simulink library "xbsIndex_r3"  (Simulink 6.1)
(part 2 of 4)

      mask prompts: num_branches "Number of Branches"; branch_length "Lengths of Branches"; explicit_period "Use Explicit Sample Period"; period "Sample Period  (use -1 to inherit first known input period)"; rst "Provide Reset Port"; en "Provide Enable Port"; dbl_ovrd "Override with Doubles"; show_param "---------------------- Show Implementation Parameters -----------------------------------------------------------------------------------"; mem_type "Memory Type"; pipeline "Pipeline to Greatest Extent Possible"; use_rpm "Use Placement Information for Core"; gen_core "Generate Core"; xl_area "FPGA Area [Slices, FFs, BRAMs, LUTs, IOBs, Emb. Mults, TBUFs]"; xl_use_area "Use Area Above For Estimation"
      mask help:
      | BLOCK IS OUT OF DATE.
      |
      | This block is from an outdated copy of the Xilinx Blockset. Please run xlUpdateModel('<model-name>') to update to the latest version.
      mask init:
      | [enPortNum,enPortStr,rstPortNum,rstPortStr] = xlport_en_rst(en,rst,3);
      | [designRoot, family, part, speed, package, simulinkPeriod, sysclkPeriod, dbl_ovrd, trimVbit] = xlSysgenSettings(gcb,1,0);
      | trimVbit=1;
      | [bg,fg] = xlcmap_r3('PayCore',dbl_ovrd);
      | iPos = get_param(gcb,'Position');
      | iWidth=iPos(3)-iPos(1); iHeight=iPos(4)-iPos(2);
      | iCx=iWidth/2;
      | iCy=iHeight/2;
      | [logoX, logoY] = xlogo(iPos);
      | 
      | % one time added for param list
      | latency = 1;
      | dblOvrd = dbl_ovrd;
      | useCore = 1;
      | precision0 = 1;
      | precision1 = 1;
      | explicitClk = explicit_period;
      | gen_core = 1;
      | rpm = use_rpm;
      | hasEN = en;
      | hasRST = rst;
      | % just pass everything to s-function
      | sfcn_mwsv__ = get_param(gcb, 'MaskWSVariables');
      | 
      | nport = get_param(gcbh, 'ports');
      | nin = nport(1);
      | nout = nport(2);
      mask Help: eval('xlWeb(xlhtmldoclink(''Interleaver Deinterleaver''))');
      mask StyleString: popup(Interleaver|Deinterleaver),edit,edit,checkbox,edit,checkbox,checkbox,checkbox,checkbox,popup(Automatically Chosen|Block RAM|Distributed RAM),checkbox,checkbox,checkbox,edit,checkbox
      mask Display:
      | patch([0 iWidth iWidth 0],[0 0 iHeight iHeight] , bg);
      | patch(logoX,logoY , fg);
      | port_label('input',1,'din');
      | port_label('output',1,'dout' );
      | port_label('output',2,'vout');
      | port_label('input',2,'vin');
      | port_label('input',enPortNum,enPortStr);
      | port_label('input',rstPortNum,rstPortStr);
      | plot([0 0 iWidth iWidth 0], [0 iHeight iHeight 0 0]);
  Inverter : S-Function  FunctionName=xldeprecated  Parameters=nin,nout  mask(Xilinx Inverter){latency=0, explicit_period=off, period=1, en=off, dbl_ovrd=off, show_param=off, xl_area=[0, 0, 0, 0, 0, 0, 0], xl_use_area=off}
      mask prompts: explicit_period "Use Explicit Sample Period"; period "Sample Period  (use -1 to inherit first known input period)"; en "Provide Enable Port"; dbl_ovrd "Override with Doubles"; show_param "---------------------- Show Implementation Parameters -----------------------------------------------------------------------------------"; xl_area "FPGA Area [Slices, FFs, BRAMs, LUTs, IOBs, Emb. Mults, TBUFs]"; xl_use_area "Use Area Above For Estimation"
      mask help:
      | BLOCK IS OUT OF DATE.
      |
      | This block is from an outdated copy of the Xilinx Blockset. Please run xlUpdateModel('<model-name>') to update to the latest version.
      mask init:
      | [enPortNum,enPortStr] = xlport_en_rst(en,0,2);
      | 
      | [designRoot, family, part, speed, package, simulinkPeriod, sysclkPeriod, dbl_ovrd, trimVbit] = xlSysgenSettings(gcb,1,1);
      | zstr=''; zpstr='';
      | if latency > 0
      |   zstr = 'z';
      |   zpstr = sprintf('-%d', latency);
      | end
      | [bg,fg] = xlcmap_r3('XBlock',dbl_ovrd);
      | iPos = get_param(gcb,'Position');
      | iWidth=iPos(3)-iPos(1); iHeight=iPos(4)-iPos(2);
      | iCx=iWidth/2;
      | iCy=iHeight/2;
      | [logoX, logoY] = xlogo(iPos);
      | zstrx = 0.45*iWidth-3; if (zstrx<3) zstrx=3; end
      | zstry = 0.36*iHeight-7; if (zstry<3) zstry=3; end
      | 
      | 
      | 
      | % one time added for param list
      | dblOvrd = dbl_ovrd;
      | precision0 = 1;
      | explicitClk = explicit_period;
      | 
      | hasEN = en;
      | 
      | % just pass everything to s-function
      | sfcn_mwsv__ = get_param(gcb, 'MaskWSVariables');
      | 
      | nport = get_param(gcbh, 'ports');
      | nin = nport(1);
      | nout = nport(2);
      mask Help: eval('xlWeb(xlhtmldoclink(''Inverter''))');
      mask Display:
      | patch([0 iWidth iWidth 0],[0 0 iHeight iHeight] , bg);
      | patch(logoX,logoY, fg);
      | text(zstrx,zstry,zstr);
      | text(zstrx+5,zstry+5,zpstr);
      | disp(' not');
      | port_label('input',enPortNum,enPortStr);
      | ;plot([0 0 iWidth iWidth 0], [0 iHeight iHeight 0 0]);
  J.83 Modulator : S-Function  FunctionName=xldeprecated  Parameters=nin,nout  mask(J.83 Modulator){}
      mask help:
      | BLOCK IS OUT OF DATE.
      |
      | This block is from an outdated copy of the Xilinx Blockset. Please run xlUpdateModel('<model-name>') to update to the latest version.
      mask init:
      | % Set Block Logo
      | [bg,fg] = xlcmap_r3('PayCore',0);
      | iPos = get_param(gcb,'Position');
      | iWidth=iPos(3)-iPos(1); iHeight=iPos(4)-iPos(2);
      | iCx=iWidth/2;
      | iCy=iHeight/2;
      | [logoX, logoY] = xlogo(iPos);
      | 
      | errormsg = ['This block has not yet been installed.  You may download this and other blocks from the Xilinx web site by clicking on the block help button.'];
      | num_inports = 0;
      | num_outports = 0;
      | nport = get_param(gcbh, 'ports');
      | nin = nport(1);
      | nout = nport(2);
      mask Help: eval('xlWeb(xlhtmldoclink(''J.83 Modulator''))');
      mask Display:
      | patch([0 iWidth iWidth 0],[0 0 iHeight iHeight] , bg);
      | patch(logoX,logoY, fg);
      | text(iCx-29,iCy,'Not Installed');
      | plot([0 0 iWidth iWidth 0], [0 iHeight iHeight 0 0]);
  LFSR : S-Function  FunctionName=xldeprecated  Parameters=nin,nout  mask(Xilinx Linear Feedback Shift Register){lfsr_type=Fibonacci, gate_type=XOR, output_type=off, n_bits=6, bin_pt=4, arith_type=Unsigned, polynomial='11', rst_value='3F', reloadable_seed=off, input_type=off, explicit_period=on, period=1, rst=off, en=off, dbl_ovrd=off, show_param=off, useSRL16s=off, use_rpm=off, gen_core=off, xl_area=[0, 0, 0, 0, 0, 0, 0], xl_use_area=off}
      mask prompts: lfsr_type "Type"; gate_type "Gate Type"; output_type "Parallel Output"; n_bits "Number of Bits in LFSR"; bin_pt "Binary Point Position"; arith_type "Arithmetic Type"; polynomial "Feedback Polynomial (Enter hex value enclosed with ticks)"; rst_value "Initial Value (Enter hex value enclosed with ticks)"; reloadable_seed "Use Reloadable Seed Values"; input_type "Parallel Input"; explicit_period "Use Explicit Sample Period"; period "Sample Period"; rst "Provide Reset Port"; en "Provide Enable Port"; dbl_ovrd "Override with Doubles"; show_param "---------------------- Show Implementation Parameters -----------------------------------------------------------------------------------"; useSRL16s "Implement with SRL16s"; use_rpm "Use Placement Information for Core"; gen_core "Generate Core"; xl_area "FPGA Area [Slices, FFs, BRAMs, LUTs, IOBs, Emb. Mults, TBUFs]"; xl_use_area "Use Area Above For Estimation"
      mask help:
      | BLOCK IS OUT OF DATE.
      |
      | This block is from an outdated copy of the Xilinx Blockset. Please run xlUpdateModel('<model-name>') to update to the latest version.
      mask init:
      | numinputs = 1;
      | dinDir = 'output';
      | dinPNum = 1;
      | dinStr = '';
      | loadDir = 'output';
      | loadPNum = 1;
      | loadStr = '';
      | 
      | if (reloadable_seed)
      |    dinStr = 'din';
      |    dinDir = 'input';
      |    dinPNum = 1;
      |    loadStr = 'load';
      |    loadDir = 'input';
      |    loadPNum = 2;
      |    numinputs = numinputs + 2;
      | end
      | 
      | [enPortNum, enPortStr, rstPortNum, rstPortStr, portDir] = xlport_en_rst(en, rst, numinputs);
      | 
      | [designRoot, family, part, speed, package, simulinkPeriod, sysclkPeriod, dbl_ovrd, trimVbit] = xlSysgenSettings(gcb,1,1);
      | [bg,fg]=xlcmap_r3('XBlock',dbl_ovrd);
      | iPos = get_param(gcb,'Position');
      | iWidth=iPos(3)-iPos(1); iHeight=iPos(4)-iPos(2);
      | iCx=iWidth/2;
      | iCy=iHeight/2;
      | [logoX, logoY] = xlogo(iPos);
      | 
      | 
      | % one time added for param list
      | dblOvrd = dbl_ovrd;
      | precision0 = 2;
      | z0 = [n_bits bin_pt arith_type  1 1];
      | hasEN = en;
      | hasRST = rst;
      | latency = 1;
      | useCore = 1;
      | explicitClk = explicit_period;
      | gen_core = 1;
      | % just pass everything to s-function
      | sfcn_mwsv__ = get_param(gcb, 'MaskWSVariables');
      | 
      | nport = get_param(gcbh, 'ports');
      | nin = nport(1);
      | nout = nport(2);
      mask Help: eval('xlWeb(xlhtmldoclink(''LFSR''))');
      mask StyleString: popup(Fibonacci|Galois),popup(XOR|XNOR),checkbox,edit,edit,popup(Unsigned|Signed  (2's comp)),edit,edit,checkbox,checkbox,checkbox,edit,checkbox,checkbox,checkbox,checkbox,checkbox,checkbox,checkbox,edit,checkbox
      mask Display:
      | patch([0 iWidth iWidth 0],[0 0 iHeight iHeight] , bg);
      | patch(logoX,logoY , fg);
      | port_label('output',1,'dout');
      | port_label(dinDir,dinPNum,dinStr);
      | port_label(loadDir,loadPNum,loadStr);
      | port_label(portDir,rstPortNum,rstPortStr);
      | port_label(portDir,enPortNum,enPortStr);
      | plot([0 0 iWidth iWidth 0], [0 iHeight iHeight 0 0]);
  Logical : S-Function  FunctionName=xldeprecated  Parameters=nin,nout  mask(Xilinx Logical Block){logical_function=AND, inputs=2, precision=Full, arith_type=Unsigned, n_bits=8, bin_pt=2, align_bp=on, latency=0, explicit_period=off, period=1, en=off, dbl_ovrd=off, show_param=off, xl_area=[0, 0, 0, 0, 0, 0, 0], xl_use_area=off}
      mask prompts: logical_function "Logical Function"; inputs "Number of Inputs"; arith_type "Output Type"; n_bits "Number of Bits"; bin_pt "Binary Point"; align_bp "Align Binary Point"; explicit_period "Use Explicit Sample Period"; period "Sample Period  (use -1 to inherit first known input period)"; en "Provide Enable Port"; dbl_ovrd "Override with Doubles"; show_param "---------------------- Show Implementation Parameters -----------------------------------------------------------------------------------"; xl_area "FPGA Area [Slices, FFs, BRAMs, LUTs, IOBs, Emb. Mults, TBUFs]"; xl_use_area "Use Area Above For Estimation"
      mask help:
      | BLOCK IS OUT OF DATE.
      |
      | This block is from an outdated copy of the Xilinx Blockset. Please run xlUpdateModel('<model-name>') to update to the latest version.
      mask init:
      | [enPortNum,enPortStr] = xlport_en_rst(en,0,inputs+2);
      | 
      | num_inputs = inputs+1;
      | [designRoot, family, part, speed, package, simulinkPeriod, sysclkPeriod, dbl_ovrd, trimVbit] = xlSysgenSettings(gcb,1,1);
      | operators = [' and'; 'nand'; '  or'; ' nor'; ' xor'; 'xnor'];
      | ostr = operators(logical_function,1:4);
      | [bg,fg] = xlcmap_r3('XBlock',dbl_ovrd);
      | iPos = get_param(gcb,'Position');
      | iWidth=iPos(3)-iPos(1); iHeight=iPos(4)-iPos(2);
      | iCx=iWidth/2;
      | iCy=iHeight/2;
      | [logoX, logoY] = xlogo(iPos);
      | zstr=''; zpstr='';
      | if latency > 0
      |   zstr = 'z';
      |   zpstr = sprintf('-%d', latency);
      | end
      | zstrx = 0.45*iWidth-3; if (zstrx<3) zstrx=3; end
      | zstry = 0.36*iHeight-7; if (zstry<3) zstry=3; end
      | 
      | % one time added for param list
      | dblOvrd = dbl_ovrd;
      | numInputs = num_inputs;
      | precision0 = precision;
      | z0 = [n_bits bin_pt arith_type 1 1 ];
      | explicitClk = explicit_period;
      | hasEN = en;
      | 
      | % just pass everything to s-function
      | sfcn_mwsv__ = get_param(gcb, 'MaskWSVariables');
      | 
      | nport = get_param(gcbh, 'ports');
      | nin = nport(1);
      | nout = nport(2);
      mask Help: eval('xlWeb(xlhtmldoclink(''Logical''))');
      mask StyleString: popup(AND|NAND|OR|NOR|XOR|XNOR),popup(2|3|4),popup(Full|User Defined),popup(Unsigned|Signed  (2's comp)),edit,edit,checkbox,edit,checkbox,edit,checkbox,checkbox,checkbox,edit,checkbox
      mask Display:
      | patch([0 iWidth iWidth 0],[0 0 iHeight iHeight] ,bg);
      | patch(logoX,logoY,  fg);
      | text(zstrx,zstry,zstr);
      | text(zstrx+5,zstry+5,zpstr);
      | disp(ostr);
      | ;plot([0 0 iWidth iWidth 0], [0 iHeight iHeight 0 0]);
      | port_label('input',enPortNum,enPortStr);
  MCode : S-Function  FunctionName=xldeprecated  Parameters=nin,nout  mask(Xilinx MCode Block){mfname=xlmax, defparams={}, suppress_output=off, hide_port_list={}, explicit_period=off, period=1, dbl_ovrd=off, show_param=off, xl_area=[0, 0, 0, 0, 0, 0, 0], xl_use_area=off}
      mask prompts: mfname "MATLAB Function"; defparams "Function Parameter Bindings (cell array, e.g., {'name', value, ...})"; suppress_output "Suppress Selected Output Ports"; hide_port_list "Output Ports to Suppress (cell array, e.g., {'name1', 'name2', ...})"; explicit_period "Use Explicit Sample Period"; period "Sample Period  (use -1 to inherit first known input period)"; dbl_ovrd "Override with Doubles"; show_param "---------------------- Show Implementation Parameters -----------------------------------------------------------------------------------"; xl_area "FPGA Area (slice, FF, BRAM, LUT, IOB, Hard Mults, TBUF)"; xl_use_area "Use Area Above For Estimation"
      mask help:
      | BLOCK IS OUT OF DATE.
      |
      | This block is from an outdated copy of the Xilinx Blockset. Please run xlUpdateModel('<model-name>') to update to the latest version.
      mask init:
      | %remove these!
      | use_rpm = 0;
      | use_core = 0;
      | clear xlmcode_maskinit;
      | if ~suppress_output
      | 	hide_port_list = {};
      | end
      | mfilename = xlFindMFile(mfname);
      | [param_names_double, param_values_double, param_names_bool, param_values_bool, error_msgs] = xlmcode_parsedefparam(defparams);
      | [numin, innums, inports, numout, outnums, outports, inname, outname] = xlmcode_maskinit(mfilename, 128, param_names_double, param_values_double, param_names_bool, param_values_bool, hide_port_list);
      | 
      | if numin==0
      |   explicitClk = 1;
      | else
      |   explicitClk = explicit_period;
      | end
      | 
      | blk = gcb;
      | visstr = get_param(blk,'MaskVisibilities');
      | var = get_param(blk,'MaskNames');
      | 
      | explicit_period_pos = find(strcmp(var,'explicit_period'));
      | period_pos = find(strcmp(var,'period'));
      | if numin==0
      |   % we need to hide the explicit_period parameter and show period
      |   visstr(explicit_period_pos) = {'off'};
      |   visstr(period_pos) = {'on'};
      | else
      |   visstr(explicit_period_pos) = {'on'};
      |   if explicit_period
      |     visstr(period_pos) = {'on'};
      |   else
      |     visstr(period_pos) = {'off'};
      |   end
      | end
      | 
      | set_param(blk, 'MaskVisibilities', visstr);
      | 
      | [designRoot, family, part, speed, package, simulinkPeriod, sysclkPeriod, dbl_ovrd, trimVbit] = xlSysgenSettings(gcb,1,1);
      | [bg,fg] = xlcmap_r3('XBlock',dbl_ovrd);
      | iPos = get_param(gcb,'Position');
      | iWidth=iPos(3)-iPos(1); iHeight=iPos(4)-iPos(2);
      | iCx=iWidth/2;
      | iCy=iHeight/2;
      | [logoX, logoY] = xlogo(iPos);
      | zstr=''; zpstr='';
      | zstr = mfname;
      | zstrx = 0.50*iWidth-3-length(mfname); if (zstrx<3) zstrx=3; end
      | zstry = 0.40*iHeight+6; if (zstry<3) zstry=3; end
      | 
      | % one time added for param list
      | latency = 0;
      | dblOvrd = dbl_ovrd;
      | numInputs = numin;
      | useCore = use_core;
      | precision0 = 1;
      | z0 = [1 0 1 1 1 ];
      | precision1 = 1;
      | precision2 = 1;
      | precision3 = 1;
      | precision4 = 1;
      | precision5 = 1;
      | precision6 = 1;
      | precision7 = 1;
      | precision8 = 1;
      | precision9 = 1;
      | precision10 = 1;
      | precision11 = 1;
      | precision12 = 1;
      | precision13 = 1;
      | precision14 = 1;
      | precision15 = 1;
      | 
      | rpm = use_rpm;
      | 
      | % mwsv_list = {'mfilename', 'designRoot', 'family', 'part', 'speed', 'package', 'simulinkPeriod', 'sysclkPeriod', 'latency', 'dblOvrd', 'trimVbit', 'numInputs', 'numout', 'useCore', 'precision0', 'z0', 'explicitClk', 'param_names_double', 'param_values_double', 'param_names_bool', 'param_values_bool', 'hide_port_list', 'period'};
      | % just pass everything to s-function
      | sfcn_mwsv__ = xlfiltermwsv(get_param(gcb, 'MaskWSVariables'), {'defparams'});
      | 
      | nport = get_param(gcbh, 'ports');
      | nin = nport(1);
      | nout = nport(2);
      mask Help: eval('xlWeb(xlhtmldoclink(''MCode''))');
      mask Display:
      | patch([0 iWidth iWidth 0],[0 0 iHeight iHeight] ,bg);
      | patch(logoX,logoY,  fg);
      | disp(mfname);
      | 
      | ;plot([0 0 iWidth iWidth 0], [0 iHeight iHeight 0 0]);
      | 
      | port_label(inname, innums(1), inports{1});
      | port_label(inname, innums(2), inports{2});
      | port_label(inname, innums(3), inports{3});
      | port_label(inname, innums(4), inports{4});
      | port_label(inname, innums(5), inports{5});
      | port_label(inname, innums(6), inports{6});
      | port_label(inname, innums(7), inports{7});
      | port_label(inname, innums(8), inports{8});
      | port_label(inname, innums(9), inports{9});
      | port_label(inname, innums(10), inports{10});
      | port_label(inname, innums(11), inports{11});
      | port_label(inname, innums(12), inports{12});
      | port_label(inname, innums(13), inports{13});
      | port_label(inname, innums(14), inports{14});
      | port_label(inname, innums(15), inports{15});
      | port_label(inname, innums(16), inports{16});
      | port_label(inname, innums(17), inports{17});
      | port_label(inname, innums(18), inports{18});
      | port_label(inname, innums(19), inports{19});
      | port_label(inname, innums(20), inports{20});
      | port_label(inname, innums(21), inports{21});
      | port_label(inname, innums(22), inports{22});
      | port_label(inname, innums(23), inports{23});
      | port_label(inname, innums(24), inports{24});
      | port_label(inname, innums(25), inports{25});
      | port_label(inname, innums(26), inports{26});
      | port_label(inname, innums(27), inports{27});
      | port_label(inname, innums(28), inports{28});
      | port_label(inname, innums(29), inports{29});
      | port_label(inname, innums(30), inports{30});
      | port_label(inname, innums(31), inports{31});
      | port_label(inname, innums(32), inports{32});
      | port_label(inname, innums(33), inports{33});
      | port_label(inname, innums(34), inports{34});
      | port_label(inname, innums(35), inports{35});
      | port_label(inname, innums(36), inports{36});
      | port_label(inname, innums(37), inports{37});
      | port_label(inname, innums(38), inports{38});
      | port_label(inname, innums(39), inports{39});
      | port_label(inname, innums(40), inports{40});
      | port_label(inname, innums(41), inports{41});
      | port_label(inname, innums(42), inports{42});
      | port_label(inname, innums(43), inports{43});
      | port_label(inname, innums(44), inports{44});
      | port_label(inname, innums(45), inports{45});
      | port_label(inname, innums(46), inports{46});
      | port_label(inname, innums(47), inports{47});
      | port_label(inname, innums(48), inports{48});
      | port_label(inname, innums(49), inports{49});
      | port_label(inname, innums(50), inports{50});
      | port_label(inname, innums(51), inports{51});
      | port_label(inname, innums(52), inports{52});
      | port_label(inname, innums(53), inports{53});
      | port_label(inname, innums(54), inports{54});
      | port_label(inname, innums(55), inports{55});
      | port_label(inname, innums(56), inports{56});
      | port_label(inname, innums(57), inports{57});
      | port_label(inname, innums(58), inports{58});
      | port_label(inname, innums(59), inports{59});
      | port_label(inname, innums(60), inports{60});
      | port_label(inname, innums(61), inports{61});
      | port_label(inname, innums(62), inports{62});
      | port_label(inname, innums(63), inports{63});
      | port_label(inname, innums(64), inports{64});
      | port_label(inname, innums(65), inports{65});
      | port_label(inname, innums(66), inports{66});
      | port_label(inname, innums(67), inports{67});
      | port_label(inname, innums(68), inports{68});
      | port_label(inname, innums(69), inports{69});
      | port_label(inname, innums(70), inports{70});
      | port_label(inname, innums(71), inports{71});
      | port_label(inname, innums(72), inports{72});
      | port_label(inname, innums(73), inports{73});
      | port_label(inname, innums(74), inports{74});
      | port_label(inname, innums(75), inports{75});
      | port_label(inname, innums(76), inports{76});
      | port_label(inname, innums(77), inports{77});
      | port_label(inname, innums(78), inports{78});
      | port_label(inname, innums(79), inports{79});
      | port_label(inname, innums(80), inports{80});
      | port_label(inname, innums(81), inports{81});
      | port_label(inname, innums(82), inports{82});
      | port_label(inname, innums(83), inports{83});
      | port_label(inname, innums(84), inports{84});
      | port_label(inname, innums(85), inports{85});
      | port_label(inname, innums(86), inports{86});
      | port_label(inname, innums(87), inports{87});
      | port_label(inname, innums(88), inports{88});
      | port_label(inname, innums(89), inports{89});
      | port_label(inname, innums(90), inports{90});
      | port_label(inname, innums(91), inports{91});
      | port_label(inname, innums(92), inports{92});
      | port_label(inname, innums(93), inports{93});
      | port_label(inname, innums(94), inports{94});
      | port_label(inname, innums(95), inports{95});
      | port_label(inname, innums(96), inports{96});
      | port_label(inname, innums(97), inports{97});
      | port_label(inname, innums(98), inports{98});
      | port_label(inname, innums(99), inports{99});
      | port_label(inname, innums(100), inports{100});
      | port_label(inname, innums(101), inports{101});
      | port_label(inname, innums(102), inports{102});
      | port_label(inname, innums(103), inports{103});
      | port_label(inname, innums(104), inports{104});
      | port_label(inname, innums(105), inports{105});
      | port_label(inname, innums(106), inports{106});
      | port_label(inname, innums(107), inports{107});
      | port_label(inname, innums(108), inports{108});
      | port_label(inname, innums(109), inports{109});
      | port_label(inname, innums(110), inports{110});
      | port_label(inname, innums(111), inports{111});
      | port_label(inname, innums(112), inports{112});
      | port_label(inname, innums(113), inports{113});
      | port_label(inname, innums(114), inports{114});
      | port_label(inname, innums(115), inports{115});
      | port_label(inname, innums(116), inports{116});
      | port_label(inname, innums(117), inports{117});
      | port_label(inname, innums(118), inports{118});
      | port_label(inname, innums(119), inports{119});
      | port_label(inname, innums(120), inports{120});
      | port_label(inname, innums(121), inports{121});
      | port_label(inname, innums(122), inports{122});
      | port_label(inname, innums(123), inports{123});
      | port_label(inname, innums(124), inports{124});
      | port_label(inname, innums(125), inports{125});
      | port_label(inname, innums(126), inports{126});
      | port_label(inname, innums(127), inports{127});
      | port_label(inname, innums(128), inports{128});
      | 
      | port_label(outname, outnums(1), outports{1});
      | port_label(outname, outnums(2), outports{2});
      | port_label(outname, outnums(3), outports{3});
      | port_label(outname, outnums(4), outports{4});
      | port_label(outname, outnums(5), outports{5});
      | port_label(outname, outnums(6), outports{6});
      | port_label(outname, outnums(7), outports{7});
      | port_label(outname, outnums(8), outports{8});
      | port_label(outname, outnums(9), outports{9});
      | port_label(outname, outnums(10), outports{10});
      | port_label(outname, outnums(11), outports{11});
      | port_label(outname, outnums(12), outports{12});
      | port_label(outname, outnums(13), outports{13});
      | port_label(outname, outnums(14), outports{14});
      | port_label(outname, outnums(15), outports{15});
      | port_label(outname, outnums(16), outports{16});
      | port_label(outname, outnums(17), outports{17});
      | port_label(outname, outnums(18), outports{18});
      | port_label(outname, outnums(19), outports{19});
      | port_label(outname, outnums(20), outports{20});
      | port_label(outname, outnums(21), outports{21});
      | port_label(outname, outnums(22), outports{22});
      | port_label(outname, outnums(23), outports{23});
      | port_label(outname, outnums(24), outports{24});
      | port_label(outname, outnums(25), outports{25});
      | port_label(outname, outnums(26), outports{26});
      | port_label(outname, outnums(27), outports{27});
      | port_label(outname, outnums(28), outports{28});
      | port_label(outname, outnums(29), outports{29});
      | port_label(outname, outnums(30), outports{30});
      | port_label(outname, outnums(31), outports{31});
      | port_label(outname, outnums(32), outports{32});
      | port_label(outname, outnums(33), outports{33});
      | port_label(outname, outnums(34), outports{34});
      | port_label(outname, outnums(35), outports{35});
      | port_label(outname, outnums(36), outports{36});
      | port_label(outname, outnums(37), outports{37});
      | port_label(outname, outnums(38), outports{38});
      | port_label(outname, outnums(39), outports{39});
      | port_label(outname, outnums(40), outports{40});
      | port_label(outname, outnums(41), outports{41});
      | port_label(outname, outnums(42), outports{42});
      | port_label(outname, outnums(43), outports{43});
      | port_label(outname, outnums(44), outports{44});
      | port_label(outname, outnums(45), outports{45});
      | port_label(outname, outnums(46), outports{46});
      | port_label(outname, outnums(47), outports{47});
      | port_label(outname, outnums(48), outports{48});
      | port_label(outname, outnums(49), outports{49});
      | port_label(outname, outnums(50), outports{50});
      | port_label(outname, outnums(51), outports{51});
      | port_label(outname, outnums(52), outports{52});
      | port_label(outname, outnums(53), outports{53});
      | port_label(outname, outnums(54), outports{54});
      | port_label(outname, outnums(55), outports{55});
      | port_label(outname, outnums(56), outports{56});
      | port_label(outname, outnums(57), outports{57});
      | port_label(outname, outnums(58), outports{58});
      | port_label(outname, outnums(59), outports{59});
      | port_label(outname, outnums(60), outports{60});
      | port_label(outname, outnums(61), outports{61});
      | port_label(outname, outnums(62), outports{62});
      | port_label(outname, outnums(63), outports{63});
      | port_label(outname, outnums(64), outports{64});
      | port_label(outname, outnums(65), outports{65});
      | port_label(outname, outnums(66), outports{66});
      | port_label(outname, outnums(67), outports{67});
      | port_label(outname, outnums(68), outports{68});
      | port_label(outname, outnums(69), outports{69});
      | port_label(outname, outnums(70), outports{70});
      | port_label(outname, outnums(71), outports{71});
      | port_label(outname, outnums(72), outports{72});
      | port_label(outname, outnums(73), outports{73});
      | port_label(outname, outnums(74), outports{74});
      | port_label(outname, outnums(75), outports{75});
      | port_label(outname, outnums(76), outports{76});
      | port_label(outname, outnums(77), outports{77});
      | port_label(outname, outnums(78), outports{78});
      | port_label(outname, outnums(79), outports{79});
      | port_label(outname, outnums(80), outports{80});
      | port_label(outname, outnums(81), outports{81});
      | port_label(outname, outnums(82), outports{82});
      | port_label(outname, outnums(83), outports{83});
      | port_label(outname, outnums(84), outports{84});
      | port_label(outname, outnums(85), outports{85});
      | port_label(outname, outnums(86), outports{86});
      | port_label(outname, outnums(87), outports{87});
      | port_label(outname, outnums(88), outports{88});
      | port_label(outname, outnums(89), outports{89});
      | port_label(outname, outnums(90), outports{90});
      | port_label(outname, outnums(91), outports{91});
      | port_label(outname, outnums(92), outports{92});
      | port_label(outname, outnums(93), outports{93});
      | port_label(outname, outnums(94), outports{94});
      | port_label(outname, outnums(95), outports{95});
      | port_label(outname, outnums(96), outports{96});
      | port_label(outname, outnums(97), outports{97});
      | port_label(outname, outnums(98), outports{98});
      | port_label(outname, outnums(99), outports{99});
      | port_label(outname, outnums(100), outports{100});
      | port_label(outname, outnums(101), outports{101});
      | port_label(outname, outnums(102), outports{102});
      | port_label(outname, outnums(103), outports{103});
      | port_label(outname, outnums(104), outports{104});
      | port_label(outname, outnums(105), outports{105});
      | port_label(outname, outnums(106), outports{106});
      | port_label(outname, outnums(107), outports{107});
      | port_label(outname, outnums(108), outports{108});
      | port_label(outname, outnums(109), outports{109});
      | port_label(outname, outnums(110), outports{110});
      | port_label(outname, outnums(111), outports{111});
      | port_label(outname, outnums(112), outports{112});
      | port_label(outname, outnums(113), outports{113});
      | port_label(outname, outnums(114), outports{114});
      | port_label(outname, outnums(115), outports{115});
      | port_label(outname, outnums(116), outports{116});
      | port_label(outname, outnums(117), outports{117});
      | port_label(outname, outnums(118), outports{118});
      | port_label(outname, outnums(119), outports{119});
      | port_label(outname, outnums(120), outports{120});
      | port_label(outname, outnums(121), outports{121});
      | port_label(outname, outnums(122), outports{122});
      | port_label(outname, outnums(123), outports{123});
      | port_label(outname, outnums(124), outports{124});
      | port_label(outname, outnums(125), outports{125});
      | port_label(outname, outnums(126), outports{126});
      | port_label(outname, outnums(127), outports{127});
      | port_label(outname, outnums(128), outports{128});
  MicroBlaze Processor : Subsystem  mask(MicroBlaze Processor){t__general=0, in_if=1, in_depths=32, out_if=1, out_depths=32, async=on, rstport=off, paramchksum=1:1:32:32:on:off:off:<empty>, procmodel=off, t__hardware=0, hw_hwcosimmodel=<empty>, hw_addsimmodel=0, t__software=0, sw_editsrccode=0ffgd, sw_compsrccode=0, xlBlockVersion=6.3}
      mask prompts: t__general "::General"; in_if "Number of Input Interfaces"; in_depths "Input FIFO Depths"; out_if "Number of Output Interfaces"; out_depths "Output FIFO Depths"; async "Use Asynchronous FIFOs"; rstport "Provide Reset Port"; paramchksum "paramchecksum"; procmodel "Provide Processor Model"; t__hardware "::Hardware"; hw_hwcosimmodel "Simulation Model"; hw_addsimmodel ":button:Add Simulation Model"; t__software "::Software"; sw_editsrccode ":button:Edit Source Code"; sw_compsrccode ":button:Compile Source Code"
      mask help:
      | Provides a MicroBlaze stub for designing peripherals that communicate with the processor using Fast Simplex Links (FSL). Current MicroBlaze implementation allows a maximum of  8 input and 8 output ports.
      |
      | Select 'Provide Processor Model' to enable use of hardware co-simulation models.
      mask init:
      | [bg,fg] = xlcmap_r3('XBlock',0);
      | iPos = get_param(gcb,'Position');
      | iWidth=iPos(3)-iPos(1); iHeight=iPos(4)-iPos(2);
      | iCx=iWidth/2;
      | iCy=iHeight/2;
      | [logoX, logoY] = xlogo(iPos);
      | [xldirectory, xlSynthTool] = xlFindTargetDir(gcb);
      | 
      | if (~strcmp(bdroot(gcs),'xbsControl_r3'))
      | 	set_param(gcb, 'LinkStatus', 'none');
      | 	xlMBCallbacks('initSubsystem');
      | end;
      settings: OpenFcn=modelName = get_param(bdroot, 'name');h = errordlg(sprintf(['This block is from an outdated copy of the Xilinx Blockset.\nPlease run xlUpdateModel(''' modelName ''') to update this design.']), 'Update Required');
      mask Help: eval('xlWeb(xlhtmldoclink(''MicroBlaze Processor''))');
      mask StyleString: edit,edit,edit,edit,edit,checkbox,checkbox,edit,checkbox,edit,popup(<empty>),edit,edit,edit,edit,edit
      mask Display:
      | patch([0 iWidth iWidth 0],[0 0 iHeight iHeight] , bg);patch(logoX,logoY , fg);plot([0 0 iWidth iWidth 0], [0 iHeight iHeight 0 0]);disp('Stub');
      | port_label('input',1,'In0_data');
      | port_label('input',2,'In0_control');
      | port_label('input',3,'In0_write');
      | port_label('input',4,'Out0_read');
      | port_label('output',1,'In0_full');
      | port_label('output',2,'Out0_data');
      | port_label('output',3,'Out0_control');
      | port_label('output',4,'Out0_exists');
  ModelSim : S-Function  FunctionName=xldeprecated  Parameters=nin,nout  mask(ModelSim HDL Co-Simulation Interface){dir=./modelsim, waveform=on, leave_open=on, skip_compile=off, custom_scripts=off, pre_comp_script=, vsim_script=, post_vsim_script=, startup_timeout=40}
      mask prompts: dir "Run Co-Simulation in Directory:"; waveform "Open Waveform Viewer"; leave_open "Leave ModelSim Open at End of Simulation"; skip_compile "Skip Compilation  (use previous results )"; custom_scripts "Add Custom Scripts"; pre_comp_script "Script to Run Before Starting Compilation:"; vsim_script "Script to Run in Place of  "vsim":"; post_vsim_script "Script to Run After "vsim":"
      mask help:
      | BLOCK IS OUT OF DATE.
      |
      | This block is from an outdated copy of the Xilinx Blockset. Please run xlUpdateModel('<model-name>') to update to the latest version.
      mask init:
      | engineDLL = 'MTICosimEng.dll';
      | binDir = xlPathToReference;
      | 
      | sim_status = get_param(bdroot,'SimulationStatus');
      | 
      | [bg,fg] = xlcmap_r3('XTool');
      | 
      | iPos = get_param(gcb,'Position');
      | iWidth=iPos(3)-iPos(1); iHeight=iPos(4)-iPos(2);
      | iCx=iWidth/2;
      | iCy=iHeight/2;
      | [logoX, logoY] = xlogo(iPos);
      | 
      | [mdlPath mdlFile mdlExt] = fileparts(get_param(bdroot,'filename'));
      | 
      | screenSize = get(0,'screensize');
      | screenSize = screenSize([3 4]);
      | 
      | % just pass everything to s-function
      | sfcn_mwsv__ = get_param(gcb, 'MaskWSVariables');
      | 
      | nport = get_param(gcbh, 'ports');
      | nin = nport(1);
      | nout = nport(2);
      mask Help: eval('xlWeb(xlhtmldoclink(''ModelSim''))');
      mask Display:
      | patch([0 iWidth iWidth 0],[0 0 iHeight iHeight] , bg);
      | patch(logoX,logoY, fg);
      | plot([0 0 iWidth iWidth 0], [0 iHeight iHeight 0 0]);
      | text(6,iHeight-11,'ModelSim');
  Mult : S-Function  FunctionName=xldeprecated  Parameters=nin,nout  mask(Xilinx Multiplier){precision=Full, arith_type=Signed  (2's comp), n_bits=8, bin_pt=2, quantization=Truncate, overflow=Wrap, latency=3, explicit_period=off, period=1, en=off, dbl_ovrd=off, show_param=off, mult_type=Parallel, oversample=2, use_embedded=off, pipeline=on, use_rpm=on, placement_style=Rectangular Shape, gen_core=off, xl_area=[0, 0, 0, 0, 0, 0, 0], xl_use_area=off}
      mask prompts: arith_type "Output Type"; n_bits "Number of Bits"; bin_pt "Binary Point"; explicit_period "Use Explicit Sample Period"; period "Sample Period  (use -1 to inherit first known input period)"; en "Provide Enable Port"; dbl_ovrd "Override with Doubles"; show_param "---------------------- Show Implementation Parameters -----------------------------------------------------------------------------------"; mult_type "Multiplier Type"; oversample "Hardware Over-Sampling Rate"; use_embedded "Use Embedded Multipliers"; pipeline "Pipeline to Greatest Extent Possible"; use_rpm "Use Placement Information for Core"; placement_style "Placement Style"; gen_core "Generate Core"; xl_area "FPGA Area [Slices, FFs, BRAMs, LUTs, IOBs, Emb. Mults, TBUFs]"; xl_use_area "Use Area Above For Estimation"
      mask help:
      | BLOCK IS OUT OF DATE.
      |
      | This block is from an outdated copy of the Xilinx Blockset. Please run xlUpdateModel('<model-name>') to update to the latest version.
      mask init:
      | rst = 0;
      | [enPortNum,enPortStr,rstPortNum,rstPortStr] = xlport_en_rst(en,rst,3);
      | multtype = mult_type;
      | if (multtype==2)
      |   osamp = oversample;
      | else
      |   osamp = 1;
      | end
      | [designRoot, family, part, speed, package, simulinkPeriod, sysclkPeriod, dbl_ovrd, trimVbit] = xlSysgenSettings(gcb,1,1);
      | zstr='';
      | zpstr='';
      | if latency > 0
      |   zstr = 'z';
      |   zpstr = sprintf('-%d', latency);
      | end
      | [bg,fg] = xlcmap_r3('XBlock',dbl_ovrd);
      | iPos = get_param(gcb,'Position');
      | iWidth=iPos(3)-iPos(1); iHeight=iPos(4)-iPos(2);
      | iCx=iWidth/2;
      | iCy=iHeight/2;
      | [logoX, logoY] = xlogo(iPos);
      | zstrx = 0.45*iWidth-3; if (zstrx<3) zstrx=3; end
      | zstry = 0.36*iHeight-7; if (zstry<3) zstry=3; end
      | 
      | % one time added for param list
      | dblOvrd = dbl_ovrd;
      | useCore = 1;
      | precision0 = precision;
      | z0 = [n_bits  bin_pt arith_type quantization overflow];
      | explicitClk = explicit_period;
      | oversample = osamp;
      | 
      | rpm = use_rpm;
      | style = placement_style;
      | hasRST = rst;
      | hasEN = en;
      | gen_core = 1;
      | % just pass everything to s-function
      | sfcn_mwsv__ = get_param(gcb, 'MaskWSVariables');
      | 
      | nport = get_param(gcbh, 'ports');
      | nin = nport(1);
      | nout = nport(2);
      mask Help: eval('xlWeb(xlhtmldoclink(''Mult''))');
      mask StyleString: popup(Full|User Defined),popup(Unsigned|Signed  (2's comp)),edit,edit,popup(Truncate|Round  (unbiased: +/- Inf)),popup(Wrap|Saturate|Flag as Error),edit,checkbox,edit,checkbox,checkbox,checkbox,popup(Parallel|Sequential),edit,checkbox,checkbox,checkbox,popup(Rectangular Shape|Triangular Packing),checkbox,edit,checkbox
      mask Display:
      | patch([0 iWidth iWidth 0],[0 0 iHeight iHeight] , bg);
      | patch(logoX,logoY, fg);
      | text(zstrx,zstry,zstr);
      | text(zstrx+5,zstry+5,zpstr);
      | port_label('input',1,'a');
      | port_label('input',2,'b');
      | port_label('output',1,'(ab)');
      | port_label('input',enPortNum,enPortStr);
      | ;plot([0 0 iWidth iWidth 0], [0 iHeight iHeight 0 0]);
  Multiple Subsystem Generator : Subsystem  Tag=xlStitcher  mask(Xilinx Subsystem Generator){}
      mask help: Double click to launch the Xilinx Multiple Subsystem Generator
      mask init:
      | [bg,fg]=xlcmap_r3('XTool');
      | iPos = get_param(gcb,'Position');
      | iWidth=iPos(3)-iPos(1); iHeight=iPos(4)-iPos(2);
      | iCx=iWidth/2;
      | iCy=iHeight/2;
      | [logoX, logoY] = xlogo(iPos);
      settings: AttributesFormatString=Multiple Subsystem\nGenerator  OpenFcn=modelName = get_param(bdroot, 'name');h = errordlg(sprintf(['This block is from an outdated copy of the Xilinx Blockset.\nPlease run xlUpdateModel(''' modelName ''') to update this design.']), 'Update Required');
      mask Help: eval('xlWeb(xlhtmldoclink(''Multiple Subsystem Generator''))');
      mask Display:
      | patch([0 iWidth iWidth 0],[0 0 iHeight iHeight] , bg);
      | patch(logoX,logoY, fg);
      | ;plot([0 0 iWidth iWidth 0], [0 iHeight iHeight 0 0]);
  Mux : S-Function  FunctionName=xldeprecated  Parameters=nin,nout  mask(Xilinx Multiplexer Block){inputs=2, precision=Full, arith_type=Signed  (2's comp), n_bits=8, bin_pt=2, quantization=Truncate, overflow=Wrap, latency=0, explicit_period=off, period=1, en=off, dbl_ovrd=off, show_param=off, mux_type=off, use_rpm=off, gen_core=off, xl_area=[0, 0, 0, 0, 0, 0, 0], xl_use_area=off}
      mask prompts: inputs "Number of Inputs"; arith_type "Arithmetic Type"; n_bits "Number of Bits"; bin_pt "Binary Point"; explicit_period "Use Explicit Sample Period"; period "Sample Period  (use -1 to inherit first known input period)"; en "Provide Enable Port"; dbl_ovrd "Override with Doubles"; show_param "---------------------- Show Implementation Parameters -----------------------------------------------------------------------------------"; mux_type "Use Tristate Buffers"; use_rpm "Use Placement Information for Core"; gen_core "Generate Core"; xl_area "FPGA Area [Slices, FFs, BRAMs, LUTs, IOBs, Emb. Mults, TBUFs]"; xl_use_area "Use Area Above For Estimation"
      mask help:
      | BLOCK IS OUT OF DATE.
      |
      | This block is from an outdated copy of the Xilinx Blockset. Please run xlUpdateModel('<model-name>') to update to the latest version.
      mask init:
      | [designRoot, family, part, speed, package, simulinkPeriod, sysclkPeriod, dbl_ovrd, trimVbit] = xlSysgenSettings(gcb,1,1);
      | num_inputs = inputs+1;
      | [bg,fg] = xlcmap_r3('XBlock',dbl_ovrd);
      | zstr='';
      | zpstr='';
      | if latency > 0
      |   zstr = 'z';
      |   zpstr = sprintf('-%d', latency);
      | end
      | 
      | dprt = [2:inputs+2 2+zeros(1,32-inputs)];
      | dstr0 = 'd0';
      | dstr1 = 'd1';
      | dstr2='';dstr3='';dstr4='';dstr5='';dstr6='';dstr7='';dstr8='';dstr9='';dstr10='';
      | dstr11='';dstr12='';dstr12='';dstr13='';dstr14='';dstr15='';dstr16='';dstr17='';dstr18='';dstr19='';dstr20='';dstr21='';dstr22='';dstr23='';dstr24='';dstr25='';dstr26='';dstr27='';dstr28='';dstr29='';dstr30='';dstr31='';
      | 
      | if (inputs>=2) dstr2 = 'd2'; end
      | if (inputs>=3) dstr3 = 'd3'; end
      | if (inputs>=4) dstr4 = 'd4'; end
      | if (inputs>=5) dstr5 = 'd5'; end
      | if (inputs>=6) dstr6 = 'd6'; end
      | if (inputs>=7) dstr7 = 'd7'; end
      | if (inputs>=8) dstr8 = 'd8'; end
      | if (inputs>=9) dstr9 = 'd9'; end
      | if (inputs>=10) dstr10 = 'd10'; end
      | if (inputs>=11) dstr11 = 'd11'; end
      | if (inputs>=12) dstr12 = 'd12'; end
      | if (inputs>=13) dstr13 = 'd13'; end
      | if (inputs>=14) dstr14 = 'd14'; end
      | if (inputs>=15) dstr15 = 'd15'; end
      | if (inputs>=16) dstr16 = 'd16'; end
      | if (inputs>=17) dstr17 = 'd17'; end
      | if (inputs>=18) dstr18 = 'd18'; end
      | if (inputs>=19) dstr19 = 'd19'; end
      | if (inputs>=20) dstr20 = 'd20'; end
      | if (inputs>=21) dstr21 = 'd21'; end
      | if (inputs>=22) dstr22 = 'd22'; end
      | if (inputs>=23) dstr23 = 'd23'; end
      | if (inputs>=24) dstr24 = 'd24'; end
      | if (inputs>=25) dstr25 = 'd25'; end
      | if (inputs>=26) dstr26 = 'd26'; end
      | if (inputs>=27) dstr27 = 'd27'; end
      | if (inputs>=28) dstr28 = 'd28'; end
      | if (inputs>=29) dstr29 = 'd29'; end
      | if (inputs>=30) dstr30 = 'd30'; end
      | if (inputs>=31) dstr31 = 'd31'; end
      | 
      | iPos = get_param(gcb,'Position');
      | iWidth=iPos(3)-iPos(1); iHeight=iPos(4)-iPos(2);
      | iCx=iWidth/2;
      | iCy=iHeight/2;
      | [logoX, logoY] = xlogo(iPos);
      | 
      | rst = 0;
      | [enPortNum, enPortStr, rstPortNum, rstPortStr, portDir] = xlport_en_rst(en, rst, num_inputs+2);
      | % one time added for param list
      | hasEN = en;
      | hasRST = rst;
      | dblOvrd = dbl_ovrd;
      | numInputs = num_inputs;
      | muxType = mux_type;
      | useCore = 1;
      | precision0 = precision;
      | z0 = [n_bits  bin_pt arith_type quantization overflow];
      | explicitClk = explicit_period;
      | gen_core = 1;
      | 
      | % just pass everything to s-function
      | sfcn_mwsv__ = get_param(gcb, 'MaskWSVariables');
      | 
      | nport = get_param(gcbh, 'ports');
      | nin = nport(1);
      | nout = nport(2);
      mask Help: eval('xlWeb(xlhtmldoclink(''Mux''))');
      mask StyleString: popup(2|3|4|5|6|7|8|9|10|11|12|13|14|15|16|17|18|19|20|21|22|23|24|25|26|27|28|29|30|31|32),popup(Full|User Defined),popup(Unsigned|Signed  (2's comp)),edit,edit,popup(Truncate|Round  (unbiased: +/- Inf)),popup(Wrap|Saturate|Flag as Error),edit,checkbox,edit,checkbox,checkbox,checkbox,checkbox,checkbox,checkbox,edit,checkbox
      mask Display:
      | patch([0 iWidth iWidth 0],[0 1/7*iHeight 6/7*iHeight iHeight] , bg);
      | patch(logoX,logoY, fg);
      | plot([0 iWidth iWidth 0 0],[0 1/7*iHeight 6/7*iHeight iHeight 0] );
      | text(iCx-5,iCy-5,zstr);
      | text(iCx,iCy,zpstr);
      | port_label('input',1,'sel');
      | port_label('input',dprt(1),dstr0);
      | port_label('input',dprt(2),dstr1);
      | port_label('input',dprt(2),dstr1);
      | port_label('input',dprt(3),dstr2);
      | port_label('input',dprt(4),dstr3);
      | port_label('input',dprt(5),dstr4);
      | port_label('input',dprt(6),dstr5);
      | port_label('input',dprt(7),dstr6);
      | port_label('input',dprt(8),dstr7);
      | port_label('input',dprt(9),dstr8);
      | port_label('input',dprt(10),dstr9);
      | port_label('input',dprt(11),dstr10);
      | port_label('input',dprt(12),dstr11);
      | port_label('input',dprt(13),dstr12);
      | port_label('input',dprt(14),dstr13);
      | port_label('input',dprt(15),dstr14);
      | port_label('input',dprt(16),dstr15);
      | port_label('input',dprt(17),dstr16);
      | port_label('input',dprt(18),dstr17);
      | port_label('input',dprt(19),dstr18);
      | port_label('input',dprt(20),dstr19);
      | port_label('input',dprt(21),dstr20);
      | port_label('input',dprt(22),dstr21);
      | port_label('input',dprt(23),dstr22);
      | port_label('input',dprt(24),dstr23);
      | port_label('input',dprt(25),dstr24);
      | port_label('input',dprt(26),dstr25);
      | port_label('input',dprt(27),dstr26);
      | port_label('input',dprt(28),dstr27);
      | port_label('input',dprt(29),dstr28);
      | port_label('input',dprt(30),dstr29);
      | port_label('input',dprt(31),dstr30);
      | port_label('input',dprt(32),dstr31);
      | port_label(portDir,enPortNum,enPortStr);
  Negate : S-Function  FunctionName=xldeprecated  Parameters=nin,nout  mask(Xilinx Negate Block){precision=Full, arith_type=Unsigned, n_bits=8, bin_pt=2, quantization=Truncate, overflow=Wrap, latency=0, explicit_period=off, period=1, en=off, dbl_ovrd=off, use_core=on, show_param=off, use_rpm=on, gen_core=off, xl_area=[0, 0, 0, 0, 0, 0, 0], xl_use_area=off}
      mask prompts: precision "Output Precision"; arith_type "Output Type"; n_bits "Number of Bits"; bin_pt "Binary Point Position"; explicit_period "Use Explicit Sample Period"; period "Sample Period  (use -1 to inherit first known input period)"; en "Provide Enable Port"; dbl_ovrd "Override with Doubles"; use_core "Implement with Xilinx Smart-IP Core  (if possible)"; show_param "---------------------- Show Implementation Parameters -----------------------------------------------------------------------------------"; use_rpm "Use Placement Information for Core"; gen_core "Generate Core"; xl_area "FPGA Area [Slices, FFs, BRAMs, LUTs, IOBs, Emb. Mults, TBUFs]"; xl_use_area "Use Area Above For Estimation"
      mask help:
      | BLOCK IS OUT OF DATE.
      |
      | This block is from an outdated copy of the Xilinx Blockset. Please run xlUpdateModel('<model-name>') to update to the latest version.
      mask init:
      | rst = 0;
      | if(latency > 0)
      |    [enPortNum,enPortStr,rstPortNum,rstPortStr] = xlport_en_rst(en,rst,2);
      | else
      |     [enPortNum,enPortStr,rstPortNum,rstPortStr] = xlport_en_rst(0,0,2);
      | end
      | [designRoot, family, part, speed, package, simulinkPeriod, sysclkPeriod, dbl_ovrd, trimVbit] = xlSysgenSettings(gcb,1,1);
      | str = 'x (-1)';
      | zstr=''; zpstr='';
      | if latency > 0
      |   zstr = 'z';
      |   zpstr = sprintf('-%d', latency);
      | end
      | [bg,fg] = xlcmap_r3('XBlock',dbl_ovrd);
      | iPos = get_param(gcb,'Position');
      | iWidth=iPos(3)-iPos(1); iHeight=iPos(4)-iPos(2);
      | iCx=iWidth/2;
      | iCy=iHeight/2;
      | [logoX, logoY] = xlogo(iPos);
      | logoX = logoX*.54 + 2;
      | logoY = logoY*.54+ iHeight*.23;
      | zstrx = 5;
      | zstry = 0.36*iHeight-7; if (zstry<3) zstry=3; end
      | 
      | % one time added for param list
      | useCore = use_core;
      | dblOvrd = dbl_ovrd;
      | precision0 = precision;
      | z0 = [n_bits bin_pt arith_type quantization overflow];
      | explicitClk = explicit_period;
      | 
      | rpm = use_rpm;
      | hasEN = en;
      | hasRST = rst;
      | gen_core = 1;
      | 
      | % just pass everything to s-function
      | sfcn_mwsv__ = get_param(gcb, 'MaskWSVariables');
      | 
      | nport = get_param(gcbh, 'ports');
      | nin = nport(1);
      | nout = nport(2);
      mask Help: eval('xlWeb(xlhtmldoclink(''Negate''))');
      mask StyleString: popup(Full|User Defined),popup(Unsigned|Signed  (2's comp)),edit,edit,popup(Truncate|Round  (unbiased: +/- Inf)),popup(Wrap|Saturate|Error),edit,checkbox,edit,checkbox,checkbox,checkbox,checkbox,checkbox,checkbox,edit,checkbox
      mask Display:
      | patch([0 iWidth 0],[0 iCy iHeight] , bg);
      | patch(logoX,logoY , fg);
      | plot([0 iWidth 0 0],[0 iCy iHeight 0] );
      | text(zstrx,zstry,zstr);
      | text(zstrx+5,zstry+5,zpstr);
      | port_label('output',1,[str '   ']);
      | port_label('input',enPortNum,enPortStr);
  Parallel to Serial : S-Function  FunctionName=xldeprecated  Parameters=nin,nout  mask(Xilinx Parallel to Serial Block){output_order=Least Significant Word First, arith_type=Unsigned, input_bits=8, output_bits=1, bin_pt=0, latency=0, explicit_period=off, period=1, en=off, dbl_ovrd=off, show_param=off, xl_area=[0, 0, 0, 0, 0, 0, 0], xl_use_area=off}
      mask prompts: output_order "Output Order"; arith_type "Output Arithmetic Type"; input_bits "Number of Input Bits"; output_bits "Number of Output Bits"; bin_pt "Output Binary Point"; explicit_period "Use Explicit Sample Period"; period "Sample Period  (use -1 to inherit first known input period)"; en "Provide Enable Port"; dbl_ovrd "Override with Doubles"; show_param "---------------------- Show Implementation Parameters -----------------------------------------------------------------------------------"; xl_area "FPGA Area [Slices, FFs, BRAMs, LUTs, IOBs, Emb. Mults, TBUFs]"; xl_use_area "Use Area Above For Estimation"
      mask help:
      | BLOCK IS OUT OF DATE.
      |
      | This block is from an outdated copy of the Xilinx Blockset. Please run xlUpdateModel('<model-name>') to update to the latest version.
      mask init:
      | rst = 0;
      | [enPortNum,enPortStr,rstPortNum,rstPortStr] = xlport_en_rst(en,rst,2);
      | 
      | [designRoot, family, part, speed, package, simulinkPeriod, sysclkPeriod, dbl_ovrd, trimVbit] = xlSysgenSettings(gcb,1,1);
      | [bg,fg] = xlcmap_r3('XBlock',dbl_ovrd);
      | iPos = get_param(gcb,'Position');
      | iWidth=iPos(3)-iPos(1); iHeight=iPos(4)-iPos(2);
      | iCx=iWidth/2;
      | iCy=iHeight/2;
      | [logoX, logoY] = xlogo(iPos);
      | 
      | 
      | 
      | % one time added for param list
      | n_bits = output_bits;
      | precision0 = 1;
      | z0 = [output_bits bin_pt arith_type 1 1 ];
      | dblOvrd = dbl_ovrd;
      | explicitClk = explicit_period;
      | 
      | hasRST = rst;
      | hasEN = en;
      | 
      | % just pass everything to s-function
      | sfcn_mwsv__ = get_param(gcb, 'MaskWSVariables');
      | 
      | nport = get_param(gcbh, 'ports');
      | nin = nport(1);
      | nout = nport(2);
      mask Help: eval('xlWeb(xlhtmldoclink(''Parallel to Serial''))');
      mask StyleString: popup(Least Significant Word First|Most Significant Word First),popup(Unsigned|Signed  (2's comp)),edit,edit,edit,edit,checkbox,edit,checkbox,checkbox,checkbox,edit,checkbox
      mask Display:
      | patch([0 iWidth iWidth 0],[0 0 iHeight iHeight] , bg);
      | port_label('input',1,'p');
      | port_label('output',1,'s');
      | patch(logoX,logoY, fg);
      | port_label('input',enPortNum,enPortStr);
      | ;plot([0 0 iWidth iWidth 0], [0 iHeight iHeight 0 0]);
  Pause Simulation : Subsystem  mask(Xilinx Pause Simulation.){}
      mask help: Pause simulation. Pauses simulation when input is nonzero.
      mask init:
      | [bg,fg] = xlcmap_r3('XTool',0);
      | iPos = get_param(gcb,'Position');
      | iWidth=iPos(3)-iPos(1); iHeight=iPos(4)-iPos(2);
      | iCx=iWidth/2;
      | iCy=iHeight/2;
      | [logoX, logoY] = xlogo(iPos);
      settings: OpenFcn=modelName = get_param(bdroot, 'name');h = errordlg(sprintf(['This block is from an outdated copy of the Xilinx Blockset.\nPlease run xlUpdateModel(''' modelName ''') to update this design.']), 'Update Required');
      mask Help: eval('xlWeb(xlhtmldoclink(''Pause Simulation''))');
      mask Display:
      | patch([0 iWidth iWidth 0],[0 0 iHeight iHeight] , bg);
      | patch(logoX,logoY , fg);
      | ;plot([0 0 iWidth iWidth 0], [0 iHeight iHeight 0 0]);
  PicoBlaze Microcontroller : S-Function  FunctionName=xldeprecated  Parameters=nin,nout  mask(Xilinx PicoBlaze Microcontroller){version=PicoBlaze 2, display_mi=off, xl_view_as=Decimal, show_param=off, xl_area=[0, 0, 0, 0, 0, 0, 0], xl_use_area=off}
      mask prompts: display_mi "Display Internal State"; xl_view_as "Display Values As"; show_param "---------------------- Show Implementation Parameters -----------------------------------------------------------------------------------"; xl_area "FPGA Area [Slices, FFs, BRAMs, LUTs, IOBs, Emb. Mults, TBUFs]"; xl_use_area "Use Area Above For Estimation"
      mask help:
      | BLOCK IS OUT OF DATE.
      |
      | This block is from an outdated copy of the Xilinx Blockset. Please run xlUpdateModel('<model-name>') to update to the latest version.
      mask init:
      | debug_mode = display_mi;
      | [designRoot, family, part, speed, package, simulinkPeriod, sysclkPeriod, dbl_ovrd, trimVbit] = xlSysgenSettings(gcb,0,1);
      | [bg,fg] = xlcmap_r3('XBlock',dbl_ovrd);
      | iPos = get_param(gcb,'Position');
      | iWidth=iPos(3)-iPos(1); iHeight=iPos(4)-iPos(2);
      | iCx=iWidth/2;
      | iCy=iHeight/2;
      | [logoX, logoY] = xlogo(iPos);
      | if(version == 1)
      | 	int_ack_port = 5;
      | 	int_ack_str = 'addr';
      | 	addr_port = 5;
      | 	addr_str = 'addr';
      | else
      | 	int_ack_port = 5;
      | 	int_ack_str = 'int_ack';
      | 	addr_port = 6;
      | 	addr_str = 'addr';
      | end
      | % one time added for param list
      | dblOvrd = dbl_ovrd;
      | precision0 = 1;
      | precision1 = 1;
      | precision2 = 1;
      | precision3 = 1;
      | precision4 = 1;
      | precision5 = 1;
      | explicitClk = 0;
      | 
      | 
      | % just pass everything to s-function
      | sfcn_mwsv__ = get_param(gcb, 'MaskWSVariables');
      | 
      | nport = get_param(gcbh, 'ports');
      | nin = nport(1);
      | nout = nport(2);
      mask Help: eval('xlWeb(xlhtmldoclink(''PicoBlaze Microcontroller''))');
      mask StyleString: popup(PicoBlaze 2|PicoBlaze 3),checkbox,popup(Decimal|Hexadecimal),checkbox,edit,checkbox
      mask Display:
      | patch([0 iWidth iWidth 0],[0 0 iHeight iHeight] , bg);
      | patch(logoX,logoY , fg);
      | port_label('input',1,'in_port');
      | port_label('input',2,'brk');
      | port_label('input',3,'rst');
      | port_label('input',4,'instr');
      | port_label('output',1,'out_port');
      | port_label('output',2,'port_id');
      | port_label('output',3,'rs');
      | port_label('output',4,'ws');
      | port_label('output',addr_port,addr_str);
      | port_label('output',int_ack_port,int_ack_str);
      | plot([0 0 iWidth iWidth 0], [0 iHeight iHeight 0 0]);
  PicoBlaze Instruction Display : Subsystem  mask(Xilinx PicoBlaze Microcontroller Instruction Display){xl_pb_inst=LOAD s6, s7, xl_pb_pc=28, xl_pb_version=Must Specify, xl_pb_disable=off}
      mask prompts: xl_pb_version "Version"; xl_pb_disable "Disable Display"
      mask help: Instruction display. Display program counter and instruction. Disabling the display allows simulation to run at normal speed.
      mask init:
      | [bg,fg] = xlcmap_r3('XTool',0);
      | iPos = get_param(gcb,'Position');
      | iWidth=iPos(3)-iPos(1); iHeight=iPos(4)-iPos(2);
      | iCx=iWidth/2;
      | iCy=iHeight/2;
      | [logoX, logoY] = xlogo(iPos);
      settings: OpenFcn=modelName = get_param(bdroot, 'name');h = errordlg(sprintf(['This block is from an outdated copy of the Xilinx Blockset.\nPlease run xlUpdateModel(''' modelName ''') to update this design.']), 'Update Required');
      mask Help: eval('xlWeb(xlhtmldoclink(''PicoBlaze Instruction Display''))');
      mask StyleString: edit,edit,popup(Must Specify|PicoBlaze 2|PicoBlaze 3),checkbox
      mask Display:
      | patch([0 iWidth iWidth 0],[0 0 iHeight iHeight] , bg);
      | patch(logoX,logoY , fg);
      | fprintf('Inst: %s\nProgCnt: %d', xl_pb_inst, xl_pb_pc);
      | port_label('input',1,'instr');
      | port_label('input',2,'addr');
      | ;plot([0 0 iWidth iWidth 0], [0 iHeight iHeight 0 0]);
  Puncture : S-Function  FunctionName=xldeprecated  Parameters=nin,nout  mask(Xilinx Puncture Block){punc_char=[1 0 0], explicit_period=off, period=1, dbl_ovrd=off}
      mask prompts: punc_char "Puncture Code"; explicit_period "Use Explicit Sample Period"; period "Sample Period"; dbl_ovrd "Override with Doubles"
      mask help:
      | BLOCK IS OUT OF DATE.
      |
      | This block is from an outdated copy of the Xilinx Blockset. Please run xlUpdateModel('<model-name>') to update to the latest version.
      mask init:
      | if  ( find((punc_char~=1) & (punc_char~=0)))
      |     punc_code = 'error';
      | else
      |  punc_code = char( (punc_char ~= 0) + 48 );
      | end;
      | [designRoot, family, part, speed, package, simulinkPeriod, sysclkPeriod, dbl_ovrd, trimVbit] = xlSysgenSettings(gcb,1,1);
      | dbl_ovrdStr = '';
      | [bg,fg]=xlcmap_r3('XBlock',dbl_ovrd);
      | iPos = get_param(gcb,'Position');
      | iWidth=iPos(3)-iPos(1); iHeight=iPos(4)-iPos(2);
      | iCx=iWidth/2;
      | iCy=iHeight/2;
      | [logoX, logoY] = xlogo(iPos);
      | 
      | 
      | % one time added for param list
      | punc_int = bin2dec(punc_code);
      | dblOvrd = dbl_ovrd;
      | precision0 = 1;
      | explicitClk = explicit_period;
      | 
      | 
      | % just pass everything to s-function
      | sfcn_mwsv__ = get_param(gcb, 'MaskWSVariables');
      | 
      | nport = get_param(gcbh, 'ports');
      | nin = nport(1);
      | nout = nport(2);
      mask Help: eval('xlWeb(xlhtmldoclink(''Puncture''))');
      mask Display:
      | patch([0 iWidth iWidth 0],[0 0 iHeight iHeight] , bg);
      | patch(logoX,logoY , fg);
      | port_label('output',1,'Puncture');
      | 
      | ;plot([0 0 iWidth iWidth 0], [0 iHeight iHeight 0 0]);
  Quantization Error : S-Function  FunctionName=xldeprecated  Parameters=nin,nout  mask(Xilinx Quantization Error Block){extraction=Quantization Error}
      mask prompts: extraction "Extract"
      mask help:
      | BLOCK IS OUT OF DATE.
      |
      | This block is from an outdated copy of the Xilinx Blockset. Please run xlUpdateModel('<model-name>') to update to the latest version.
      mask init:
      | if (extraction==1)
      |   plabel = 'err';
      | else
      |   plabel = 'exp';
      | end
      | 
      | [bg,fg] = xlcmap_r3('IO');
      | iPos = get_param(gcb,'Position');
      | iWidth=iPos(3)-iPos(1); iHeight=iPos(4)-iPos(2);
      | iCx=iWidth/2;
      | iCy=iHeight/2;
      | [logoX, logoY] = xlogo(iPos);
      | 
      | nport = get_param(gcbh, 'ports');
      | nin = nport(1);
      | nout = nport(2);
      mask Help: eval('xlWeb(xlhtmldoclink(''Quantization Error''))');
      mask StyleString: popup(Quantization Error|Expected Value)
      mask Display:
      | patch([0 iWidth iWidth 0],[0 0 iHeight iHeight] , bg);
      | patch(logoX,logoY , fg);
      | port_label('output',1,plabel);
      | 
      | plot([0 0 iWidth iWidth 0], [0 iHeight iHeight 0 0]);
  ROM : S-Function  FunctionName=xldeprecated  Parameters=nin,nout  mask(Xilinx Single Port Read-Only Memory){depth=16, initVector=sin(pi*(0:15)/16), arith_type=Signed  (2's comp), n_bits=8, bin_pt=6, latency=1, init_zero=on, explicit_period=off, period=1, rst=off, init_reg=0, en=off, dbl_ovrd=off, show_param=off, distributed_mem=off, use_rpm=off, gen_core=off, xl_area=[0, 0, 0, 0, 0, 0, 0], xl_use_area=off}
      mask prompts: initVector "Initial Value Vector"; arith_type "Word Type"; n_bits "Number of Bits"; bin_pt "Binary Point"; init_zero "Zero Initial Output  (otherwise NaN)"; explicit_period "Use Explicit Sample Period"; period "Sample Period  (use -1 to inherit first known input period)"; rst "Provide Reset Port for Output Register"; init_reg "Initial Value for Output Register"; en "Provide Enable Port"; dbl_ovrd "Override with Doubles"; show_param "---------------------- Show Implementation Parameters -----------------------------------------------------------------------------------"; distributed_mem "Use Distributed Memory (instead of block RAM)"; use_rpm "Use Placement Information for Core"; gen_core "Generate Core"; xl_area "FPGA Area [Slices, FFs, BRAMs, LUTs, IOBs, Emb. Mults, TBUFs]"; xl_use_area "Use Area Above For Estimation"
      mask help:
      | BLOCK IS OUT OF DATE.
      |
      | This block is from an outdated copy of the Xilinx Blockset. Please run xlUpdateModel('<model-name>') to update to the latest version.
      mask init:
      | [designRoot, family, part, speed, package, simulinkPeriod, sysclkPeriod, dbl_ovrd, trimVbit] = xlSysgenSettings(gcb,1,1);
      | if isempty(family)
      | 	family = 'Virtex2';
      | end;
      | [bg,fg] = xlcmap_r3('XBlock',dbl_ovrd);
      | iPos = get_param(gcb,'Position');
      | iWidth=iPos(3)-iPos(1); iHeight=iPos(4)-iPos(2);
      | iCx=iWidth/2;
      | iCy=iHeight/2;
      | [logoX, logoY] = xlogo(iPos);
      | 
      | if (arith_type==1)
      |   bool = 1;
      | else
      |   bool = 0;
      |   arith_type=arith_type-1;
      | end
      | 
      | if(distributed_mem==0)
      | 	hasRST = rst;
      | else
      | 	init_reg = 0;
      | 	rst = 0;
      | end
      | 
      | [enPortNum,enPortStr,rstPortNum,rstPortStr] = xlport_en_rst(en,rst,2);
      | % one time added for param list
      | hasEN = en;
      | dblOvrd = dbl_ovrd;
      | useCore = 1;
      | z0 = [n_bits bin_pt arith_type 1 1];
      | precision0 = 2;
      | init = initVector;
      | initZero = init_zero;
      | distributed = distributed_mem;
      | explicitClk = explicit_period;
      | gen_core = 1;
      | rpm = use_rpm;
      | 
      | % just pass everything to s-function
      | sfcn_mwsv__ = get_param(gcb, 'MaskWSVariables');
      | 
      | nport = get_param(gcbh, 'ports');
      | nin = nport(1);
      | nout = nport(2);
      mask Help: eval('xlWeb(xlhtmldoclink(''ROM''))');
      mask StyleString: edit,edit,popup(Boolean|Unsigned|Signed  (2's comp)),edit,edit,edit,checkbox,checkbox,edit,checkbox,edit,checkbox,checkbox,checkbox,checkbox,checkbox,checkbox,edit,checkbox
      mask Display:
      | patch([0 iWidth iWidth 0],[0 0 iHeight iHeight] , bg);
      | patch(logoX,logoY , fg);
      | port_label('input',1,'addr');
      | port_label('input',enPortNum,enPortStr);
      | port_label('input',rstPortNum,rstPortStr);
      | 
      | ;plot([0 0 iWidth iWidth 0], [0 iHeight iHeight 0 0]);
  RS Decoder : S-Function  FunctionName=xldeprecated  Parameters=nin,nout  mask(Xilinx Reed-Solomon Decoder){code_spec=Custom, sym_width=8, nn=204, kk=188, poly_char=[ 1 0 0 0 1 1 1 0 1], gen_start=0, scale=1, hasStart=off, hasErase=off, explicit_period=off, period=1, rst=off, dbl_ovrd=off, show_param=off, use_rpm=on, gen_core=off, xl_area=[0, 0, 0, 0, 0, 0, 0], xl_use_area=off}
      mask prompts: code_spec "Code Specification"; sym_width "Symbol Width (integer between 3 and 12)"; nn "n (number of symbols per code block)"; kk "k (number of information symbols per code block)"; poly_char "Field Polynomial (example: [ 1 0 1 1]  =>  x^3  +  x  +  1)"; gen_start "Generator Start (log of first root of generator polynomial)"; scale "Scaling Factor for Generator Polynomial"; hasStart "Provide Start Pin"; hasErase "Enable Erasure Decoding"; explicit_period "Use Explicit Sample Period"; period "Sample Period  (use -1 to inherit first known input period)"; rst "Provide Reset Port"; dbl_ovrd "Override with Doubles"; show_param "---------------------- Show Implementation Parameters -----------------------------------------------------------------------------------"; use_rpm "Use Placement Information for Core"; gen_core "Generate Core"; xl_area "FPGA Area [Slices, FFs, BRAMs, LUTs, IOBs, Emb. Mults, TBUFs]"; xl_use_area "Use Area Above For Estimation"
      mask help:
      | BLOCK IS OUT OF DATE.
      |
      | This block is from an outdated copy of the Xilinx Blockset. Please run xlUpdateModel('<model-name>') to update to the latest version.
      mask init:
      | if  ( find((poly_char~=1) & (poly_char~=0)))
      |     poly = 'error';
      | else
      |   poly = char( (poly_char ~= 0) + 48 );
      | end;
      | if(code_spec == 2)
      |    sym_width = 8;
      |    nn = 207;
      |    kk = 187;
      |    poly = '100011101';
      |    gen_start = 0;
      |    scale = 1;
      | elseif(code_spec == 3)
      |    sym_width = 8;
      |    poly = '110000111';
      |    gen_start = 112;
      |    scale = 11;
      | elseif(code_spec == 4)
      |    sym_width = 8;
      |    nn = 204;
      |    kk = 188;
      |    poly = '100011101';
      |    gen_start = 0;
      |    scale = 1;
      | elseif(code_spec == 5)
      |    sym_width = 8;
      |    nn = 126;
      |    kk = 112;
      |    poly = '110000111';
      |    gen_start = 120;
      |    scale = 1;
      | elseif(code_spec == 6)
      |    sym_width = 8;
      |    nn = 194;
      |    kk = 178;
      |    poly = '110000111';
      |    gen_start = 120;
      |    scale = 1;
      | elseif(code_spec == 7)
      |    sym_width = 8;
      |    nn = 208;
      |    kk = 192;
      |    poly = '110000111';
      |    gen_start = 120;
      |    scale = 1;
      | elseif(code_spec == 8)
      |    sym_width = 8;
      |    nn = 219;
      |    kk = 201;
      |    poly = '110000111';
      |    gen_start = 120;
      |    scale = 1;
      | elseif(code_spec == 9)
      |    sym_width = 8;
      |    nn = 225;
      |    kk = 205;
      |    poly = '110000111';
      |    gen_start = 120;
      |    scale = 1;
      | end
      | 
      | numinputs = 3;
      | startPNum = 1;
      | startStr = '';
      | erasePNum = 1;
      | eraseStr = '';
      | erasecntPNum = 1;
      | erasecntStr = '';
      | if (hasStart)
      |   startStr = 'start';
      |   startPNum = numinputs;
      |   numinputs = numinputs + 1;
      |   if (hasErase)
      |      eraseStr = 'erase';
      |      erasePNum = numinputs;
      |      numinputs = numinputs + 1;
      |      erasecntPNum = 6;
      |      erasecntStr = 'erase_cnt';
      |  end
      | else
      |  if (hasErase)
      |      eraseStr = 'erase';
      |      erasePNum = numinputs;
      |      numinputs = numinputs + 1;
      |      erasecntPNum = 6;
      |      erasecntStr = 'erase_cnt';
      |    end
      | end
      | [enPortNum, enPortStr, rstPortNum, rstPortStr, portDir] = xlport_en_rst(0, rst, numinputs);
      | dstr = sprintf('(%d,\n%d)',nn,kk);
      | [designRoot, family, part, speed, package, simulinkPeriod, sysclkPeriod, dbl_ovrd, trimVbit] = xlSysgenSettings(gcb,1,0);
      | trimVbit=1;
      | [bg,fg] = xlcmap_r3('PayCore',dbl_ovrd);
      | iPos = get_param(gcb,'Position');
      | iWidth=iPos(3)-iPos(1); iHeight=iPos(4)-iPos(2);
      | iCx=iWidth/2;
      | iCy=iHeight/2;
      | [logoX, logoY] = xlogo(iPos);
      | 
      | % one time added for param list
      | alpha = bin2dec(poly);
      | hasRST = rst;
      | latency = 2;
      | dblOvrd = dbl_ovrd;
      | useCore = 1;
      | precision0 = 1;
      | precision1 = 1;
      | precision2 = 1;
      | precision3 = 1;
      | precision4 = 1;
      | precision5 = 1;
      | explicitClk = explicit_period;
      | 
      | gen_core =1 ;
      | % just pass everything to s-function
      | sfcn_mwsv__ = get_param(gcb, 'MaskWSVariables');
      | 
      | 
      | nport = get_param(gcbh, 'ports');
      | nin = nport(1);
      | nout = nport(2);
      mask Help: eval('xlWeb(xlhtmldoclink(''RS Decoder''))');
      mask StyleString: popup(Custom|ATSC|CCSDS|DVB|IESS-308 (126)|IESS-308 (194)|IESS-308 (208)|IESS-308 (219)|IESS-308 (225)),edit,edit,edit,edit,edit,edit,checkbox,checkbox,checkbox,edit,checkbox,checkbox,checkbox,checkbox,checkbox,edit,checkbox
      mask Display:
      | patch([0 iWidth iWidth 0],[0 0 iHeight iHeight] , bg);
      | patch(logoX,logoY , fg);
      | text(iCx/1.4-10,iCy+2,dstr);
      | port_label('output',1,'dout' );
      | port_label('output',2,'vout' );
      | port_label('output',3,'info' );
      | port_label('output',4,'fail' );
      | port_label('output',5,'err_cnt' );
      | port_label('output',erasecntPNum,erasecntStr);
      | port_label('input',1,'din');
      | port_label('input',2,'vin');
      | port_label('input',startPNum,startStr);
      | port_label('input',erasePNum,eraseStr);
      | port_label(portDir,rstPortNum,rstPortStr);
      | plot([0 0 iWidth iWidth 0], [0 iHeight iHeight 0 0]);
  RS Encoder : S-Function  FunctionName=xldeprecated  Parameters=nin,nout  mask(Xilinx Reed-Solomon Encoder){code_spec=Custom, sym_width=8, nn=204, kk=188, poly_char=[ 1 0 0 0 1 1 1 0 1], gen_start=0, scale=1, hasStart=off, explicit_period=off, period=1, rst=off, dbl_ovrd=off, show_param=off, use_rpm=on, gen_core=off, xl_area=[0, 0, 0, 0, 0, 0, 0], xl_use_area=off}
      mask prompts: code_spec "Code Specification"; sym_width "Symbol Width (integer between 3 and 12)"; nn "n (number of symbols per code block)"; kk "k (number of information symbols per code block)"; poly_char "Field Polynomial (example: [ 1 0 1 1]  => x^3  +  x  +  1)"; gen_start "Generator Start (log of first root of generator polynomial)"; scale "Scaling Factor for Generator Polynomial"; hasStart "Provide Start and Bypass Pins"; explicit_period "Use Explicit Sample Period"; period "Sample Period  (use -1 to inherit first known input period)"; rst "Provide Reset Port"; dbl_ovrd "Override with Doubles"; show_param "---------------------- Show Implementation Parameters -----------------------------------------------------------------------------------"; use_rpm "Use Placement Information for Core"; gen_core "Generate Core"; xl_area "FPGA Area [Slices, FFs, BRAMs, LUTs, IOBs, Emb. Mults, TBUFs]"; xl_use_area "Use Area Above For Estimation"
      mask help:
      | BLOCK IS OUT OF DATE.
      |
      | This block is from an outdated copy of the Xilinx Blockset. Please run xlUpdateModel('<model-name>') to update to the latest version.
      mask init:
      | if  (find((poly_char~=1) & (poly_char~=0)))
      |     poly = 'error';
      | else
      |   poly = char( (poly_char ~= 0) + 48 );
      | end;
      | if(code_spec == 2)
      |    sym_width = 8;
      |    nn = 207;
      |    kk = 187;
      |    poly = '100011101';
      |    gen_start = 0;
      |    scale = 1;
      | elseif(code_spec == 3)
      |    sym_width = 8;
      |    poly = '110000111';
      |    gen_start = 112;
      |    scale = 11;
      | elseif(code_spec == 4)
      |    sym_width = 8;
      |    nn = 204;
      |    kk = 188;
      |    poly = '100011101';
      |    gen_start = 0;
      |    scale = 1;
      | elseif(code_spec == 5)
      |    sym_width = 8;
      |    nn = 126;
      |    kk = 112;
      |    poly = '110000111';
      |    gen_start = 120;
      |    scale = 1;
      | elseif(code_spec == 6)
      |    sym_width = 8;
      |    nn = 194;
      |    kk = 178;
      |    poly = '110000111';
      |    gen_start = 120;
      |    scale = 1;
      | elseif(code_spec == 7)
      |    sym_width = 8;
      |    nn = 208;
      |    kk = 192;
      |    poly = '110000111';
      |    gen_start = 120;
      |    scale = 1;
      | elseif(code_spec == 8)
      |    sym_width = 8;
      |    nn = 219;
      |    kk = 201;
      |    poly = '110000111';
      |    gen_start = 120;
      |    scale = 1;
      | elseif(code_spec == 9)
      |    sym_width = 8;
      |    nn = 225;
      |    kk = 205;
      |    poly = '110000111';
      |    gen_start = 120;
      |    scale = 1;
      | end
      | 
      | numinputs = 3;
      | startPNum = 1;
      | startStr = '';
      | bypassPNum = 1;
      | bypassStr = '';
      | if (hasStart)
      |   startStr = 'start';
      |   startPNum = numinputs;
      |   numinputs = numinputs + 1;
      |   bypassPNum = numinputs;
      |   numinputs = numinputs + 1;
      |   bypassStr = 'bypass';
      | end
      | [enPortNum, enPortStr, rstPortNum, rstPortStr, portDir] = xlport_en_rst(0, rst, numinputs);
      | dstr = sprintf('(%d,\n%d)',nn,kk);
      | [designRoot, family, part, speed, package, simulinkPeriod, sysclkPeriod, dbl_ovrd, trimVbit] = xlSysgenSettings(gcb,1,0);
      | trimVbit=1;
      | [bg,fg] = xlcmap_r3('PayCore',dbl_ovrd);
      | iPos = get_param(gcb,'Position');
      | iWidth=iPos(3)-iPos(1); iHeight=iPos(4)-iPos(2);
      | iCx=iWidth/2;
      | iCy=iHeight/2;
      | [logoX, logoY] = xlogo(iPos);
      | 
      | % one time added for param list
      | alpha = bin2dec(poly);
      | hasRST = rst;
      | latency = 1;
      | dblOvrd = dbl_ovrd;
      | useCore = 1;
      | precision0 = 1;
      | precision1 = 1;
      | precision2 = 1;
      | precision3 = 1;
      | explicitClk = explicit_period;
      | 
      | gen_core = 1;
      | % just pass everything to s-function
      | sfcn_mwsv__ = get_param(gcb, 'MaskWSVariables');
      | 
      | 
      | nport = get_param(gcbh, 'ports');
      | nin = nport(1);
      | nout = nport(2);
      mask Help: eval('xlWeb(xlhtmldoclink(''RS Encoder''))');
      mask StyleString: popup(Custom|ATSC|CCSDS|DVB|IESS-308 (126)|IESS-308 (194)|IESS-308 (208)|IESS-308 (219)|IESS-308 (225)),edit,edit,edit,edit,edit,edit,checkbox,checkbox,edit,checkbox,checkbox,checkbox,checkbox,checkbox,edit,checkbox
      mask Display:
      | patch([0 iWidth iWidth 0],[0 0 iHeight iHeight] , bg);
      | patch(logoX,logoY , fg);
      | text(iCx/1.4-10,iCy+2,dstr);
      | port_label('output',1,'dout' );
      | port_label('output',2,'vout' );
      | port_label('output',3,'info' );
      | port_label('output',4,'rfd' );
      | port_label('input',1,'din');
      | port_label('input',2,'vin');
      | port_label('input',startPNum,startStr);
      | port_label('input',bypassPNum,bypassStr);
      | port_label(portDir,rstPortNum,rstPortStr);
      | plot([0 0 iWidth iWidth 0], [0 iHeight iHeight 0 0]);
  Register : S-Function  FunctionName=xldeprecated  Parameters=nin,nout  mask(Xilinx Register Block){init=0, reg_only_valid=off, explicit_period=off, period=1, rst=off, en=off, out_en=off, dbl_ovrd=off, show_param=off, xl_area=[0, 0, 0, 0, 0, 0, 0], xl_use_area=off}
      mask prompts: init "Initial Value"; reg_only_valid "Register Only Valid Data"; explicit_period "Use Explicit Sample Period"; period "Sample Period  (use -1 to inherit first known input period)"; rst "Provide Reset Port"; en "Provide Enable Port"; out_en "Propagate Enable Sample Period"; dbl_ovrd "Override with Doubles"; show_param "---------------------- Show Implementation Parameters -----------------------------------------------------------------------------------"; xl_area "FPGA Area [Slices, FFs, BRAMs, LUTs, IOBs, Emb. Mults, TBUFs]"; xl_use_area "Use Area Above For Estimation"
      mask help:
      | BLOCK IS OUT OF DATE.
      |
      | This block is from an outdated copy of the Xilinx Blockset. Please run xlUpdateModel('<model-name>') to update to the latest version.
      mask init:
      | [designRoot, family, part, speed, package, simulinkPeriod, sysclkPeriod, dbl_ovrd, trimVbit] = xlSysgenSettings(gcb,1,1);
      | rstPortNum = 1;
      | rstPortStr = '';
      | enPortNum = 1;
      | enPortStr =  '';
      | if (rst)
      |     rstPortNum = 2;
      |     rstPortStr = 'rst';
      | end
      | if ((rst == 0) & (en == 1))
      |     enPortNum = 2;
      |     enPortStr = 'en';
      | end
      | if ((rst == 1) & (en == 1))
      |     enPortNum = 3;
      |     enPortStr = 'en';
      | end
      | [bg,fg] = xlcmap_r3('XBlock',dbl_ovrd);
      | iPos = get_param(gcb,'Position');
      | iWidth=iPos(3)-iPos(1); iHeight=iPos(4)-iPos(2);
      | iCx=iWidth/2;
      | iCy=iHeight/2;
      | [logoX, logoY] = xlogo(iPos);
      | zstr='z'; zpstr='-1';
      | zstrx = iCx-3; if (zstrx<16) zstr='';zpstr=''; end
      | zstry = iCy;
      | 
      | 
      | 
      | % one time added for param list
      | precision0 = 1;
      | latency = 1;
      | dblOvrd = dbl_ovrd;
      | vOnly = reg_only_valid;
      | explicitClk = explicit_period;
      | hasRST = rst;
      | hasEN = en;
      | 
      | 
      | % just pass everything to s-function
      | sfcn_mwsv__ = get_param(gcb, 'MaskWSVariables');
      | 
      | nport = get_param(gcbh, 'ports');
      | nin = nport(1);
      | nout = nport(2);
      mask Help: eval('xlWeb(xlhtmldoclink(''Register''))');
      mask Display:
      | patch([0 iWidth iWidth 0],[0 0 iHeight iHeight] , bg);
      | patch(logoX,logoY, fg);
      | text(zstrx,zstry,zstr);
      | text(zstrx+5,zstry+5,zpstr);
      | port_label('input',1,'d');
      | port_label('input',rstPortNum,rstPortStr);
      | port_label('input',enPortNum,enPortStr);
      | port_label('output',1,'q' );
      | ;plot([0 0 iWidth iWidth 0], [0 iHeight iHeight 0 0]);
  Reinterpret : S-Function  FunctionName=xldeprecated  Parameters=nin,nout  mask(Xilinx Type Reinterpreting Block){force_arith_type=on, arith_type=Unsigned, force_bin_pt=on, bin_pt=0, force_valid=on}
      mask prompts: force_arith_type "Force Arithmetic Type"; arith_type "Output Arithmetic Type"; force_bin_pt "Force Binary Point Position"; bin_pt "Output Binary Point"; force_valid "Force Output Valid"
      mask help:
      | BLOCK IS OUT OF DATE.
      |
      | This block is from an outdated copy of the Xilinx Blockset. Please run xlUpdateModel('<model-name>') to update to the latest version.
      mask init:
      | [designRoot, family, part, speed, package, simulinkPeriod, sysclkPeriod, dbl_ovrd, trimVbit] = xlSysgenSettings(gcb,0,2);
      | dbl_ovrd = 0;
      | ostr = 'no-op';
      | if (force_arith_type | force_bin_pt|force_valid)
      |   ostr = 'force';
      | end
      | [bg,fg] = xlcmap_r3('XBlock',dbl_ovrd);
      | iPos = get_param(gcb,'Position');
      | iWidth=iPos(3)-iPos(1); iHeight=iPos(4)-iPos(2);
      | iCx=iWidth/2;
      | iCy=iHeight/2;
      | [logoX, logoY] = xlogo(iPos);
      | zstrx = 0.45*iWidth-11; if (zstrx<3) zstrx=3; end
      | zstry = 0.36*iHeight-7; if (zstry<3) zstry=3; end
      | 
      | 
      | % one time added for param list
      | latency = 0;
      | dblOvrd = dbl_ovrd;
      | precision0 = 1;
      | chg_arith_type = force_arith_type;
      | chg_binpt = force_bin_pt;
      | new_arith_type = arith_type;
      | new_binpt = bin_pt;
      | 
      | 
      | % just pass everything to s-function
      | sfcn_mwsv__ = get_param(gcb, 'MaskWSVariables');
      | 
      | nport = get_param(gcbh, 'ports');
      | nin = nport(1);
      | nout = nport(2);
      mask Help: eval('xlWeb(xlhtmldoclink(''Reinterpret''))');
      mask StyleString: checkbox,popup(Unsigned|Signed  (2's comp)),checkbox,edit,checkbox
      mask Display:
      | patch([0 iWidth iWidth 0],[0 0 iHeight iHeight] , bg);
      | patch(logoX,logoY , fg);
      | port_label('output',1,ostr);
      | plot([0 0 iWidth iWidth 0], [0 iHeight iHeight 0 0]);
  Relational : S-Function  FunctionName=xldeprecated  Parameters=nin,nout  mask(Xilinx Relational Block){mode=a=b, latency=1, explicit_period=off, period=1, en=off, dbl_ovrd=off, show_param=off, xl_area=[0, 0, 0, 0, 0, 0, 0], xl_use_area=off}
      mask prompts: mode "Comparison:"; explicit_period "Use Explicit Sample Period"; period "Sample Period  (use -1 to inherit first known input period)"; en "Provide Enable Port"; dbl_ovrd "Override with Doubles"; show_param "---------------------- Show Implementation Parameters -----------------------------------------------------------------------------------"; xl_area "FPGA Area [Slices, FFs, BRAMs, LUTs, IOBs, Emb. Mults, TBUFs]"; xl_use_area "Use Area Above For Estimation"
      mask help:
      | BLOCK IS OUT OF DATE.
      |
      | This block is from an outdated copy of the Xilinx Blockset. Please run xlUpdateModel('<model-name>') to update to the latest version.
      mask init:
      | [enPortNum,enPortStr] = xlport_en_rst(en,0,3);
      | 
      | [designRoot, family, part, speed, package, simulinkPeriod, sysclkPeriod, dbl_ovrd, trimVbit] = xlSysgenSettings(gcb,1,1);
      | zstr='';
      | zpstr='';
      | if latency > 0
      |   zstr = 'z';
      |   zpstr = sprintf('-%d', latency);
      | end
      | [bg,fg] = xlcmap_r3('XBlock',dbl_ovrd);
      | iPos = get_param(gcb,'Position');
      | iWidth=iPos(3)-iPos(1); iHeight=iPos(4)-iPos(2);
      | iCx=iWidth/2;
      | iCy=iHeight/2;
      | [logoX, logoY] = xlogo(iPos);
      | if mode == 1
      |   str = 'a=b';
      | elseif mode == 2
      |   str = 'a!=b';
      | elseif mode == 3
      |   str = 'a<b';
      | elseif mode == 4
      |   str = 'a>b';
      | elseif mode == 5
      |   str = 'a<=b';
      | elseif mode == 6
      |   str = 'a >=b';
      | end
      | zstrx = 0.45*iWidth-3; if (zstrx<3) zstrx=3; end
      | zstry = 0.36*iHeight-7; if (zstry<3) zstry=3; end
      | 
      | 
      | % one time added for param list
      | dblOvrd = dbl_ovrd;
      | precision0 = 1;
      | explicitClk = explicit_period;
      | 
      | hasEN = en;
      | 
      | % just pass everything to s-function
      | sfcn_mwsv__ = get_param(gcb, 'MaskWSVariables');
      | 
      | nport = get_param(gcbh, 'ports');
      | nin = nport(1);
      | nout = nport(2);
      mask Help: eval('xlWeb(xlhtmldoclink(''Relational''))');
      mask StyleString: popup(a=b|a!=b|a<b|a>b|a<=b|a>=b),edit,checkbox,edit,checkbox,checkbox,checkbox,edit,checkbox
      mask Display:
      | patch([0 iWidth iWidth 0],[0 0 iHeight iHeight] , bg);
      | patch(logoX,logoY, fg);
      | text(zstrx,zstry,zstr);
      | text(zstrx+5,zstry+5,zpstr);
      | port_label('input',1,'a');
      | port_label('input',2,'b');
      | port_label('output',1,str );
      | port_label('input',enPortNum,enPortStr);
      | ;plot([0 0 iWidth iWidth 0], [0 iHeight iHeight 0 0]);
  Resource Estimator : Subsystem  Tag=resEstTag  mask(Xilinx Resource Estimator Block){xl_estimator_area=[0, 0, 0, 0, 0, 0, 0], xl_use_estimator_area=off, simulink_period=1, mrp_directory=D:/matlabR12/toolbox/xilinx/sysgen/bin}
      mask prompts: xl_estimator_area "FPGA Area [Slices, FFs, BRAMs, LUTs, IOBs, Mults, TBUFs]"; xl_use_estimator_area "Use Above Area For Estimation"; simulink_period "Simulink Period"; mrp_directory "Map Report Directory"
      mask help: When used in a subsystem, or top level system, an estimation of the resources used in this (sub)system can be done by choosing an estimation type. Double click on the icon to access these features.
      mask init:
      | [bg, fg] = xlcmap_r3('XTool');
      | 
      | %[bg1, fg] = xlcmap_r3('XBlock',0);
      | iPos = get_param(gcb,'Position');
      | iWidth=iPos(3)-iPos(1); iHeight=iPos(4)-iPos(2);
      | iCx=iWidth/2;
      | iCy=iHeight/2;
      | [logoX, logoY] = xlogo(iPos);
      | 
      | %xlEstimateResources('XL_INITIALIZE_GUI');
      settings: AttributesFormatString=Resource\nEstimator  OpenFcn=modelName = get_param(bdroot, 'name');h = errordlg(sprintf(['This block is from an outdated copy of the Xilinx Blockset.\nPlease run xlUpdateModel(''' modelName ''') to update this design.']), 'Update Required');
      mask Help: eval('xlWeb(xlhtmldoclink(''Resource Estimator''))');
      mask Display:
      | patch([0 iWidth iWidth 0],[0 0 iHeight iHeight] , bg);
      | patch(logoX,logoY , fg);
      | ;plot([0 0 iWidth iWidth 0], [0 iHeight iHeight 0 0]);
  Sample Time : S-Function  FunctionName=xldeprecated  Parameters=nin,nout  mask(Xilinx Sample Time Reporter){}
      mask help:
      | BLOCK IS OUT OF DATE.
      |
      | This block is from an outdated copy of the Xilinx Blockset. Please run xlUpdateModel('<model-name>') to update to the latest version.
      mask init:
      | [designRoot, family, part, speed, package, simulinkPeriod, sysclkPeriod, dbl_ovrd, trimVbit] = xlSysgenSettings(gcb,0,0);
      | [bg,fg] = xlcmap_r3('IO');
      | iPos = get_param(gcb,'Position');
      | iWidth=iPos(3)-iPos(1); iHeight=iPos(4)-iPos(2);
      | iCx=iWidth/2;
      | iCy=iHeight/2;
      | shapeX = iCx* (1 + cos(0:pi/6:2*pi));
      | shapeY = iCy* (1 + sin(0:pi/6:2*pi));
      | 
      | 
      | 
      | % one time added for param list
      | 
      | 
      | % just pass everything to s-function
      | sfcn_mwsv__ = get_param(gcb, 'MaskWSVariables');
      | 
      | nport = get_param(gcbh, 'ports');
      | nin = nport(1);
      | nout = nport(2);
      mask Help: eval('xlWeb(xlhtmldoclink(''Sample Time''))');
      mask Display:
      | patch(shapeX,shapeY, bg);
      | plot(shapeX,shapeY);
      | disp('ST');
  Scale : S-Function  FunctionName=xldeprecated  Parameters=nin,nout  mask(Xilinx Scaling Block){scale_factor=4, explicit_period=off, period=1, dbl_ovrd=off}
      mask prompts: scale_factor "Scale Factor  (power of two by which to scale input)"; explicit_period "Use Explicit Sample Period"; period "Sample Period"; dbl_ovrd "Override with Doubles"
      mask help:
      | BLOCK IS OUT OF DATE.
      |
      | This block is from an outdated copy of the Xilinx Blockset. Please run xlUpdateModel('<model-name>') to update to the latest version.
      mask init:
      | [designRoot, family, part, speed, package, simulinkPeriod, sysclkPeriod, dbl_ovrd, trimVbit] = xlSysgenSettings(gcb,1,1);
      | pstr = sprintf('%d', scale_factor);
      | [bg,fg] = xlcmap_r3('XBlock',dbl_ovrd);
      | iPos = get_param(gcb,'Position');
      | iWidth=iPos(3)-iPos(1); iHeight=iPos(4)-iPos(2);
      | iCx=iWidth/2;
      | iCy=iHeight/2;
      | [logoX, logoY] = xlogo(iPos);
      | logoX = logoX*.54 + 2;
      | logoY = logoY*.54+ iHeight*.23;
      | 
      | 
      | % one time added for param list
      | precision0 = 1;
      | dblOvrd = dbl_ovrd;
      | explicitClk = explicit_period;
      | 
      | 
      | % just pass everything to s-function
      | sfcn_mwsv__ = get_param(gcb, 'MaskWSVariables');
      | 
      | nport = get_param(gcbh, 'ports');
      | nin = nport(1);
      | nout = nport(2);
      mask Help: eval('xlWeb(xlhtmldoclink(''Scale''))');
      mask Display:
      | patch([0 iWidth 0],[0 iCy iHeight] , bg);
      | patch(logoX,logoY , fg);
      | plot([0 iWidth 0 0],[0 iCy iHeight 0] );
      | text(iCx-20,iCy-3,'x 2');
      | text(iCx-6,iCy+3,pstr);
  Serial to Parallel : S-Function  FunctionName=xldeprecated  Parameters=nin,nout  mask(Xilinx Serial to Parallel Block){input_order=Least Significant Word First, arith_type=Unsigned, input_bits=1, output_bits=8, bin_pt=2, latency=1, explicit_period=off, period=1, en=off, dbl_ovrd=off, show_param=off, xl_area=[0, 0, 0, 0, 0, 0, 0], xl_use_area=off}
      mask prompts: input_order "Input Order"; arith_type "Output Arithmetic Type"; input_bits "Number of Input Bits"; output_bits "Number of Output Bits"; bin_pt "Binary Point"; explicit_period "Use Explicit Sample Period"; period "Sample Period  (use -1 to inherit first known input period)"; en "Provide Enable Port"; dbl_ovrd "Override with Doubles"; show_param "---------------------- Show Implementation Parameters -----------------------------------------------------------------------------------"; xl_area "FPGA Area [Slices, FFs, BRAMs, LUTs, IOBs, Emb. Mults, TBUFs]"; xl_use_area "Use Area Above For Estimation"
      mask help:
      | BLOCK IS OUT OF DATE.
      |
      | This block is from an outdated copy of the Xilinx Blockset. Please run xlUpdateModel('<model-name>') to update to the latest version.
      mask init:
      | rst = 0;
      | [enPortNum,enPortStr,rstPortNum,rstPortStr] = xlport_en_rst(en,rst,2);
      | 
      | [designRoot, family, part, speed, package, simulinkPeriod, sysclkPeriod, dbl_ovrd, trimVbit] = xlSysgenSettings(gcb,1,1);
      | [bg,fg] = xlcmap_r3('XBlock',dbl_ovrd);
      | iPos = get_param(gcb,'Position');
      | iWidth=iPos(3)-iPos(1); iHeight=iPos(4)-iPos(2);
      | iCx=iWidth/2;
      | iCy=iHeight/2;
      | [logoX, logoY] = xlogo(iPos);
      | 
      | % one time added for param list
      | precision0 = 2;
      | z0 = [output_bits bin_pt arith_type 1 1 ];
      | n_bits = output_bits;
      | dblOvrd = dbl_ovrd;
      | explicitClk = explicit_period;
      | 
      | hasRST = rst;
      | hasEN = en;
      | 
      | % just pass everything to s-function
      | sfcn_mwsv__ = get_param(gcb, 'MaskWSVariables');
      | 
      | nport = get_param(gcbh, 'ports');
      | nin = nport(1);
      | nout = nport(2);
      mask Help: eval('xlWeb(xlhtmldoclink(''Serial to Parallel''))');
      mask StyleString: popup(Least Significant Word First|Most Significant Word First),popup(Unsigned|Signed  (2's comp)),edit,edit,edit,edit,checkbox,edit,checkbox,checkbox,checkbox,edit,checkbox
      mask Display:
      | patch([0 iWidth iWidth 0],[0 0 iHeight iHeight] , bg);
      | patch(logoX,logoY, fg);
      | port_label('input',1,'s');
      | port_label('output',1,'p');
      | port_label('input',enPortNum,enPortStr);
      | ;plot([0 0 iWidth iWidth 0], [0 iHeight iHeight 0 0]);
  Shared Memory : S-Function  FunctionName=xldeprecated  Parameters=nin,nout  mask(Xilinx Shared Memory Random Access Memory){shared_memory_name='Bar', depth=16, arith_type=Unsigned, n_bits=0, bin_pt=0, ownership=Locally Owned and Initialized, initVector=sin(pi*(0:15)/16), implementation=Block RAM, mutex=Unprotected, mode=Read and Write, write_mode=Read After Write, time_out=0, explicit_period=off, period=1, use_rpm=off, show_param=off, xl_area=[0, 0, 0, 0, 0, 0, 0], xl_use_area=off}
      mask prompts: shared_memory_name "Shared Memory Name"; arith_type "Arithmetic Type"; n_bits "Number of Output Bits"; bin_pt "Binary Point Position"; ownership "Ownership and Initialization"; initVector "Initial Value Vector"; mutex "Access Protection"; mode "Access Mode"; write_mode "Write Mode"; time_out "Memory Access Timeout (sec)"; explicit_period "Use Explicit Sample Period"; period "Sample Period  (use -1 to inherit first known input period)"; use_rpm "Use Placement Information for Core"; show_param "---------------------- Show Implementation Parameters -----------------------------------------------------------------------------------"; xl_area "FPGA Area [Slices, FFs, BRAMs, LUTs, IOBs, Emb. Mults, TBUFs]"; xl_use_area "Use Area Above For Estimation"
      mask help:
      | BLOCK IS OUT OF DATE.
      |
      | This block is from an outdated copy of the Xilinx Blockset. Please run xlUpdateModel('<model-name>') to update to the latest version.
      mask init:
      | if (ownership==1) % Locally owned
      | 	create_memory = 1;
      | else
      | 	create_memory = 0;
      | end
      | 
      | if (implementation==1)
      | 	distributed_mem = 0;
      | else
      | 	distributed_mem = 1;
      | end
      | 
      | [designRoot, family, part, speed, package, simulinkPeriod, sysclkPeriod, dbl_ovrd, trimVbit] = xlSysgenSettings(gcb,0,1);
      | 
      | if isempty(family)
      | 	family = 'Virtex2';
      | end;
      | 
      | if(strcmp(time_out, 'Inf') | strcmp(time_out,'INF'))
      | 	time_out = -1.0;
      | end;
      | 
      | [bg,fg] = xlcmap_r3('Shmem',0);
      | iPos = get_param(gcb,'Position');
      | iWidth=iPos(3)-iPos(1); iHeight=iPos(4)-iPos(2);
      | iCx=iWidth/2;
      | iCy=iHeight/2;
      | [logoX, logoY] = xlogo(iPos);
      | 
      | latency = 1;
      | hasRst = 0;
      | hasEn = 0;
      | init_zero = 1;
      | init_reg = 0;
      | rst = 0;
      | en = 0;
      |  
      | switch (mode)
      |   case 1 % RW
      |     dinPortNum = 2;
      |     dinPortStr = 'din';
      |     wePortNum = 3;
      |     wePortStr = 'we';
      |     doutPortNum = 1;
      |     doutPortStr = 'dout';
      |     doutPortDir = 'output';
      |     icount = 3;
      |     ocount = 1;
      |   case 2 % RO
      |     dinPortNum = 1;
      |     dinPortStr = '';
      |     wePortNum = 1;
      |     wePortStr = '';
      |     doutPortNum = 1;
      |     doutPortStr = 'dout';
      |     doutPortDir = 'output';
      |     icount = 1;
      |     ocount = 1;
      |   case 3 % WO
      |     dinPortNum = 2;
      |     dinPortStr = 'din';
      |     wePortNum = 3;
      |     wePortStr = 'we';
      |     doutPortNum = 1;
      |     doutPortStr = '';
      |     doutPortDir = 'input';
      |     icount = 3;
      |     ocount = 0;
      | end
      | 
      | if (mutex==1)
      |   reqPortNum = icount+1;
      |   reqPortStr = 'req';
      |   grantPortNum = ocount+1;
      |   grantPortStr = 'grant';
      |   grantPortDir = 'output';
      | else
      |   reqPortNum = 1;
      |   reqPortStr = '';
      |   grantPortNum = 1;
      |   grantPortStr = '';
      |   grantPortDir = 'input';
      | end
      | 
      | % one time added for param list
      | dblOvrd = 0;
      | precision0 = 1;
      | precision1 = 1;
      | init = initVector;
      | initZero = init_zero;
      | distributed = distributed_mem;
      | explicitClk = explicit_period;
      | rpm = use_rpm;
      | 
      | % just pass everything to s-function
      | sfcn_mwsv__ = get_param(gcb, 'MaskWSVariables');
      | 
      | nport = get_param(gcbh, 'ports');
      | nin = nport(1);
      | nout = nport(2);
      settings: AttributesFormatString=<< %<shared_memory_name> >>
      mask Help: eval('xlWeb(xlhtmldoclink(''Shared Memory''))');
      mask StyleString: edit,edit,popup(Unsigned|Signed  (2's comp)),edit,edit,popup(Locally Owned and Initialized|Owned and Initialized Elsewhere),edit,popup(Block RAM|Distributed RAM),popup(Lockable|Unprotected),popup(Read and Write|Read Only|Write Only),popup(Read After Write|Read Before Write|No Read On Write),edit,checkbox,edit,checkbox,checkbox,edit,checkbox
      mask Display:
      | patch([0 iWidth iWidth 0],[0 0 iHeight iHeight] , bg);
      | patch(logoX,logoY , fg);
      | port_label('input',1,'addr');
      | port_label('input',dinPortNum,dinPortStr);
      | port_label('input',wePortNum,wePortStr);
      | port_label('input',reqPortNum,reqPortStr);
      | port_label(doutPortDir,doutPortNum,doutPortStr);
      | port_label(grantPortDir,grantPortNum,grantPortStr);
      | port_label(doutPortDir,doutPortNum,doutPortStr);
      | ;plot([0 0 iWidth iWidth 0], [0 iHeight iHeight 0 0]);
  Shared Memory Read : S-Function  Priority=20  FunctionName=xldeprecated  Parameters=nin,nout  mask(Xilinx Shared Memory Read Block){shmem_name='Bar', isFrame=off, dataType=int8, outDims=[1 1], sample_time=1, shmem_depth=0, shmem_word=0}
      mask prompts: shmem_name "Shared Memory Name"; isFrame "Use Frame-based Output (otherwise sample-based)"; dataType "Output Data Type"; outDims "Output Dimensions ( N or [M,N] )"; sample_time "Sample Time"; shmem_depth "Shared Memory Depth"; shmem_word "Shared Memory Word Size"
      mask help:
      | BLOCK IS OUT OF DATE.
      |
      | This block is from an outdated copy of the Xilinx Blockset. Please run xlUpdateModel('<model-name>') to update to the latest version.
      mask init:
      | %[designRoot, family, part, speed, package, simulinkPeriod, sysclkPeriod, dbl_ovrd, trimVbit] = xlSysgenSettings(gcb,1,2);
      | [fg,bg]=xlcmap_r3('IO',0);
      | iPos = get_param(gcb,'Position');
      | iWidth=iPos(3)-iPos(1); iHeight=iPos(4)-iPos(2);
      | iCx=iWidth/2;
      | iCy=iHeight/2;
      | [logoX, logoY] = xlogo(iPos);
      | 
      | nport = get_param(gcbh, 'ports');
      | nin = nport(1);
      | nout = nport(2);
      settings: AttributesFormatString=<< %<shmem_name> >>
      mask Help: eval('xlWeb(xlhtmldoclink(''Shared Memory Read''))');
      mask StyleString: edit,checkbox,popup(int8|uint8|int16|uint16|int32|uint32),edit,edit,edit,edit
      mask Display:
      | patch([0 iWidth iWidth 0],[0 0 iHeight iHeight] , bg);
      | patch(logoX,logoY , fg);
      | port_label('output',1,'d');
      | ;plot([0 0 iWidth iWidth 0], [0 iHeight iHeight 0 0]);
      | fprintf('depth: %d\nwidth: %d',shmem_depth,shmem_word);
  Shared Memory Write : S-Function  Priority=10  FunctionName=xldeprecated  Parameters=nin,nout  mask(Xilinx Shared Memory Block Write){shmem_name='Bar', shmem_depth=0, shmem_word=0}
      mask prompts: shmem_name "Shared Memory Name"; shmem_depth "Shared Memory Depth"; shmem_word "Shared Memory Word Size"
      mask help:
      | BLOCK IS OUT OF DATE.
      |
      | This block is from an outdated copy of the Xilinx Blockset. Please run xlUpdateModel('<model-name>') to update to the latest version.
      mask init: same as xbsIndex_r3/Shared Memory Read
      settings: AttributesFormatString=<< %<shmem_name> >>
      mask Help: eval('xlWeb(xlhtmldoclink(''Shared Memory Write''))');
      mask Display:
      | patch([0 iWidth iWidth 0],[0 0 iHeight iHeight] , bg);
      | patch(logoX,logoY , fg);
      | port_label('input',1,'d');
      | ;plot([0 0 iWidth iWidth 0], [0 iHeight iHeight 0 0]);
      | fprintf('depth: %d\nwidth: %d',shmem_depth,shmem_word);
  Shift : S-Function  FunctionName=xldeprecated  Parameters=nin,nout  mask(Xilinx Shift Block){shift_dir=Left, shift_bits=2, precision=Full, arith_type=Signed  (2's comp), n_bits=8, bin_pt=2, quantization=Truncate, overflow=Wrap, latency=0, explicit_period=off, period=1, en=off, dbl_ovrd=off, show_param=off, xl_area=[0, 0, 0, 0, 0, 0, 0], xl_use_area=off}
      mask prompts: shift_dir "Shift Direction"; shift_bits "Number of Bits"; arith_type "Output Type"; n_bits "Number of Bits"; bin_pt "Binary Point"; explicit_period "Use Explicit Sample Period"; period "Sample Period  (use -1 to inherit first known input period)"; en "Provide Enable Port"; dbl_ovrd "Override with Doubles"; show_param "---------------------- Show Implementation Parameters -----------------------------------------------------------------------------------"; xl_area "FPGA Area [Slices, FFs, BRAMs, LUTs, IOBs, Emb. Mults, TBUFs]"; xl_use_area "Use Area Above For Estimation"
      mask help:
      | BLOCK IS OUT OF DATE.
      |
      | This block is from an outdated copy of the Xilinx Blockset. Please run xlUpdateModel('<model-name>') to update to the latest version.
      mask init:
      | rst = 0;
      | if(latency > 0)
      |    [enPortNum,enPortStr,rstPortNum,rstPortStr] = xlport_en_rst(en,rst,2);
      | else
      |     [enPortNum,enPortStr,rstPortNum,rstPortStr] = xlport_en_rst(0,0,2);
      | end
      | [designRoot, family, part, speed, package, simulinkPeriod, sysclkPeriod, dbl_ovrd, trimVbit] = xlSysgenSettings(gcb,1,1);
      | zstr='';
      | zpstr='';
      | if latency > 0
      |   zstr = 'z';
      |   zpstr = sprintf('-%d', latency);
      | end
      | act_shift = (2*shift_dir-3) * shift_bits;
      | if (act_shift<0)
      |   sstr = sprintf('X << %d ', -act_shift);
      | else
      |   sstr = sprintf('X >> %d ', act_shift);
      | end
      | [bg,fg] = xlcmap_r3('XBlock', dbl_ovrd);
      | iPos = get_param(gcb,'Position');
      | iWidth=iPos(3)-iPos(1); iHeight=iPos(4)-iPos(2);
      | iCx=iWidth/2;
      | iCy=iHeight/2;
      | [logoX, logoY] = xlogo(iPos);
      | zstrx = 0.45*iWidth-15; if (zstrx<3) zstrx=3; end
      | zstry = 0.36*iHeight-7; if (zstry<3) zstry=3; end
      | 
      | % one time added for param list
      | dblOvrd = dbl_ovrd;
      | precision0 = precision;
      | z0 = [n_bits  bin_pt arith_type quantization overflow];
      | shiftDir = shift_dir;
      | shiftBits = shift_bits;
      | explicitClk = explicit_period;
      | 
      | hasEN = en;
      | hasRST = rst;
      | % just pass everything to s-function
      | sfcn_mwsv__ = get_param(gcb, 'MaskWSVariables');
      | 
      | nport = get_param(gcbh, 'ports');
      | nin = nport(1);
      | nout = nport(2);
      mask Help: eval('xlWeb(xlhtmldoclink(''Shift''))');
      mask StyleString: popup(Left|Right),edit,popup(Full|User Defined),popup(Unsigned|Signed  (2's comp)),edit,edit,popup(Truncate|Round  (unbiased: +/- Inf)),popup(Wrap|Saturate|Flag as Error),edit,checkbox,edit,checkbox,checkbox,checkbox,edit,checkbox
      mask Display:
      | patch([0 iWidth iWidth 0],[0 0 iHeight iHeight] , bg);
      | patch(logoX,logoY, fg);
      | text(zstrx,zstry,zstr);
      | text(zstrx+5,zstry+5,zpstr);
      | port_label('output',1, sstr);
      | port_label('input',enPortNum,enPortStr);
      | ;plot([0 0 iWidth iWidth 0], [0 iHeight iHeight 0 0]);
  Simulation Multiplexer : S-Function  FunctionName=xldeprecated  Parameters=nin,nout  mask(Xilinx Simulation Multiplexer){sim_sel=1, hw_sel=2}
      mask prompts: sim_sel "For Simulation,  Pass Through Data from Input Port:   (1 or 2)"; hw_sel "For Generation,  Pass Through Data from Input Port:   (1 or 2)"
      mask help:
      | BLOCK IS OUT OF DATE.
      |
      | This block is from an outdated copy of the Xilinx Blockset. Please run xlUpdateModel('<model-name>') to update to the latest version.
      mask init:
      | [designRoot, family, part, speed, package, simulinkPeriod, sysclkPeriod, dbl_ovrd, trimVbit] = xlSysgenSettings(gcb,0,0);
      | 
      | [bg, fg] = xlcmap_r3('XBlock');
      | 
      | iPos = get_param(gcb,'Position');
      | iWidth=iPos(3)-iPos(1); iHeight=iPos(4)-iPos(2);
      | iCx=iWidth/2;
      | iCy=iHeight/2;
      | [logoX, logoY] = xlogo(iPos);
      | 
      | swLineX = [0 .5 .75 1]*iWidth;
      | if (sim_sel==1)
      | 	simSwLineY = [.72 .72 .47 .47]*iHeight;
      | else
      | 	simSwLineY = [.22 .22 .47 .47]*iHeight;
      | end
      | 
      | if (hw_sel==1)
      | 	hwSwLineY = [.72 .72 .47 .47]*iHeight;
      | else
      | 	hwSwLineY = [.22 .22 .47 .47]*iHeight;
      | end
      | 
      | 
      | 
      | 
      | % one time added for param list
      | precision0 = 1;
      | latency = 0;
      | dblOvrd = 0;
      | explicitClk = 0;
      | 
      | 
      | % just pass everything to s-function
      | sfcn_mwsv__ = get_param(gcb, 'MaskWSVariables');
      | 
      | nport = get_param(gcbh, 'ports');
      | nin = nport(1);
      | nout = nport(2);
      mask Help: eval('xlWeb(xlhtmldoclink(''Simulation Multiplexer''))');
      mask Display:
      | patch([0 iWidth iWidth 0],[0 0 iHeight iHeight] , bg);
      | patch(logoX,logoY , fg);
      | plot([0 0 iWidth iWidth 0], [0 iHeight iHeight 0 0]);
      | color('red');
      | plot(swLineX,simSwLineY);
      | color('black');
      | plot(swLineX,hwSwLineY);
  SineCosine : S-Function  FunctionName=xldeprecated  Parameters=nin,nout  mask(Xilinx Sine/Cosine Block){mode=Sine, neg_sin=off, neg_cos=off, n_bits=8, latency=2, sym_output=off, explicit_period=off, period=1, en=off, dbl_ovrd=off, show_param=off, mem_type=Distributed Memory, pipeline=off, use_rpm=on, gen_core=off, xl_area=[0, 0, 0, 0, 0, 0, 0], xl_use_area=off}
      mask prompts: mode "Function"; neg_sin "Negative Sine"; neg_cos "Negative Cosine"; n_bits "Output Width"; sym_output "Symmetric Output"; explicit_period "Use Explicit Sample Period"; period "Sample Period  (use -1 to inherit first known input period)"; en "Provide Enable Port"; dbl_ovrd "Override with Doubles"; show_param "---------------------- Show Implementation Parameters -----------------------------------------------------------------------------------"; mem_type "Memory Type"; pipeline "Pipeline to Greatest Extent Possible"; use_rpm "Use Placement Information for Core"; gen_core "Generate Core"; xl_area "FPGA Area [Slices, FFs, BRAMs, LUTs, IOBs, Emb. Mults, TBUFs]"; xl_use_area "Use Area Above For Estimation"
      mask help:
      | BLOCK IS OUT OF DATE.
      |
      | This block is from an outdated copy of the Xilinx Blockset. Please run xlUpdateModel('<model-name>') to update to the latest version.
      mask init:
      | rst = 0;
      | if(latency > 0)
      |    [enPortNum,enPortStr,rstPortNum,rstPortStr] = xlport_en_rst(en,rst,2);
      | else
      |     [enPortNum,enPortStr,rstPortNum,rstPortStr] = xlport_en_rst(0,0,2);
      | end
      | [designRoot, family, part, speed, package, simulinkPeriod, sysclkPeriod, dbl_ovrd, trimVbit] = xlSysgenSettings(gcb,1,1);
      | if(sym_output == 1)
      |   bin_pt = n_bits - 2;
      | else
      |   bin_pt = n_bits-1;
      | end
      | if (neg_sin==0)
      |   sstr = 'sin';
      |  else
      |   sstr = '-sin';
      | end
      | if (neg_cos==0)
      |   cstr = 'cos';
      |  else
      |    cstr = '-cos';
      | end
      | mprt=1; mstr='';ostr2='';
      | if (mode==1)  ostr=sstr; end;
      | if (mode==2)  ostr=cstr; end;
      | if (mode==3)  mprt=2; ostr=sstr; ostr2=cstr; end;
      | 
      | [bg,fg] = xlcmap_r3('XBlock',dbl_ovrd);
      | iPos = get_param(gcb,'Position');
      | iWidth=iPos(3)-iPos(1); iHeight=iPos(4)-iPos(2);
      | iCx=iWidth/2;
      | iCy=iHeight/2;
      | [logoX, logoY] = xlogo(iPos);
      | zstrx = 0.45*iWidth-3; if (zstrx<3) zstrx=3; end
      | zstry = 0.36*iHeight-7; if (zstry<3) zstry=3; end
      | 
      | 
      | % one time added for param list
      | dblOvrd = dbl_ovrd;
      | explicitClk = explicit_period;
      | memtype = mem_type;
      | precision0 = 2;
      | z0 = [n_bits bin_pt 2 2 2];
      | useCore = 1;
      | pipelined = pipeline;
      | negsine = neg_sin;
      | negcos = neg_cos;
      | precision1 = 2;
      | z1 = [n_bits bin_pt 2 2 2];
      | hasEN = en;
      | hasRST = rst;
      | gen_core = 1;
      | 
      | % just pass everything to s-function
      | sfcn_mwsv__ = get_param(gcb, 'MaskWSVariables');
      | 
      | nport = get_param(gcbh, 'ports');
      | nin = nport(1);
      | nout = nport(2);
      mask Help: eval('xlWeb(xlhtmldoclink(''SineCosine''))');
      mask StyleString: popup(Sine|Cosine|Sine and Cosine),checkbox,checkbox,edit,edit,checkbox,checkbox,edit,checkbox,checkbox,checkbox,popup(Distributed Memory|Block RAM),checkbox,checkbox,checkbox,edit,checkbox
      mask Display:
      | patch([0 iWidth iWidth 0],[0 0 iHeight iHeight] , bg);
      | patch(logoX,logoY , fg);
      | port_label('output',1,ostr);
      | port_label('output',mprt,ostr2);
      | port_label('input',1,'theta');
      | port_label('input',enPortNum,enPortStr);
      | plot([0 0 iWidth iWidth 0], [0 iHeight iHeight 0 0]);
  Single Port RAM : S-Function  FunctionName=xldeprecated  Parameters=nin,nout  mask(Xilinx Single Port Random Access Memory){depth=16, initVector=sin(pi*(0:15)/16), write_mode=Read After Write, latency=1, init_zero=on, explicit_period=off, period=1, rst=off, init_reg=0, en=off, dbl_ovrd=off, show_param=off, distributed_mem=off, use_rpm=off, gen_core=off, xl_area=[0, 0, 0, 0, 0, 0, 0], xl_use_area=off}
      mask prompts: initVector "Initial Value Vector"; write_mode "Write Mode"; init_zero "Zero Initial Output  (otherwise NaN)"; explicit_period "Use Explicit Sample Period"; period "Sample Period  (use -1 to inherit first known input period)"; rst "Provide Reset Port for Output Register"; init_reg "Initial Value for Output Register"; en "Provide Enable Port"; dbl_ovrd "Override with Doubles"; show_param "---------------------- Show Implementation Parameters -----------------------------------------------------------------------------------"; distributed_mem "Use Distributed Memory (instead of block RAM)"; use_rpm "Use Placement Information for Core"; gen_core "Generate Core"; xl_area "FPGA Area [Slices, FFs, BRAMs, LUTs, IOBs, Emb. Mults, TBUFs]"; xl_use_area "Use Area Above For Estimation"
      mask help:
      | BLOCK IS OUT OF DATE.
      |
      | This block is from an outdated copy of the Xilinx Blockset. Please run xlUpdateModel('<model-name>') to update to the latest version.
      mask init:
      | [designRoot, family, part, speed, package, simulinkPeriod, sysclkPeriod, dbl_ovrd, trimVbit] = xlSysgenSettings(gcb,1,1);
      | if isempty(family)
      | 	family = 'Virtex2';
      | end;
      | 
      | [bg,fg] = xlcmap_r3('XBlock',dbl_ovrd);
      | iPos = get_param(gcb,'Position');
      | iWidth=iPos(3)-iPos(1); iHeight=iPos(4)-iPos(2);
      | iCx=iWidth/2;
      | iCy=iHeight/2;
      | [logoX, logoY] = xlogo(iPos);
      | [memX,memY] = memplot(iPos,min(depth,floor(iWidth/4)));
      | 
      |  
      | if(distributed_mem==0)
      | 	hasRST = rst;
      | else
      | 	init_reg = 0;
      | 	rst = 0;
      | end
      | 
      | [enPortNum,enPortStr,rstPortNum,rstPortStr] = xlport_en_rst(en,rst,4);
      | % one time added for param list
      | hasEN = en;
      | useCore = 1;
      | dblOvrd = dbl_ovrd;
      | useCore = 1;
      | precision0 = 1;
      | init = initVector;
      | initZero = init_zero;
      | distributed = distributed_mem;
      | explicitClk = explicit_period;
      | gen_core = 1;
      | rpm = use_rpm;
      | 
      | % just pass everything to s-function
      | sfcn_mwsv__ = get_param(gcb, 'MaskWSVariables');
      | 
      | nport = get_param(gcbh, 'ports');
      | nin = nport(1);
      | nout = nport(2);
      mask Help: eval('xlWeb(xlhtmldoclink(''Single Port RAM''))');
      mask StyleString: edit,edit,popup(Read After Write|Read Before Write|No Read On Write),edit,checkbox,checkbox,edit,checkbox,edit,checkbox,checkbox,checkbox,checkbox,checkbox,checkbox,edit,checkbox
      mask Display:
      | patch([0 iWidth iWidth 0],[0 0 iHeight iHeight] , bg);
      | patch(logoX,logoY , fg);
      | port_label('input',1,'addr');
      | port_label('input',2,'data');
      | port_label('input',3,'we');
      | port_label('input',enPortNum,enPortStr);
      | port_label('input',rstPortNum,rstPortStr);
      | port_label('output',1,'');
      | ;plot([0 0 iWidth iWidth 0], [0 iHeight iHeight 0 0]);
  Single-Step Simulation : Subsystem  mask(Xilinx Single-Step Simulation.){xl_status=Single-Step, xl_state=0}
      mask help: Single-Step Simulation. Double-clicking toggles between single-step simulation and continuous running mode.
      mask init:
      | [bg,fg] = xlcmap_r3('XTool',0);
      | iPos = get_param(gcb,'Position');
      | iWidth=iPos(3)-iPos(1); iHeight=iPos(4)-iPos(2);
      | iCx=iWidth/2;
      | iCy=iHeight/2;
      | [logoX, logoY] = xlogo(iPos);
      settings: OpenFcn=modelName = get_param(bdroot, 'name');h = errordlg(sprintf(['This block is from an outdated copy of the Xilinx Blockset.\nPlease run xlUpdateModel(''' modelName ''') to update this design.']), 'Update Required');
      mask Help: eval('xlWeb(xlhtmldoclink(''Single-Step Simulation''))');
      mask Display:
      | patch([0 iWidth iWidth 0],[0 0 iHeight iHeight] , bg);
      | patch(logoX,logoY , fg);
      | fprintf('%s', xl_status);
      | ;plot([0 0 iWidth iWidth 0], [0 iHeight iHeight 0 0]);
  Slice : S-Function  FunctionName=xldeprecated  Parameters=nin,nout  mask(Xilinx Slice Block){mode=Upper Bit Location + Width, nbits=1, bit1=0, base1=MSB of Input, bit0=0, base0=LSB of Input, boolean_output=off, explicit_period=off, period=1, dbl_ovrd=off}
      mask prompts: mode "Specify Range As"; nbits "Width of Slice (number of bits)"; bit1 "Offset of Top Bit"; base1 "Relative To"; bit0 "Offset of Bottom Bit"; base0 "Relative To"; boolean_output "Boolean Output"; explicit_period "Use Explicit Sample Period"; period "Sample Period"; dbl_ovrd "Override with Doubles"
      mask help:
      | BLOCK IS OUT OF DATE.
      |
      | This block is from an outdated copy of the Xilinx Blockset. Please run xlUpdateModel('<model-name>') to update to the latest version.
      mask init:
      | [designRoot, family, part, speed, package, simulinkPeriod, sysclkPeriod, dbl_ovrd, trimVbit] = xlSysgenSettings(gcb,1,1);
      | dbl_ovrdStr = '';
      | [bg,fg]=xlcmap_r3('XBlock',dbl_ovrd);
      | iPos = get_param(gcb,'Position');
      | iWidth=iPos(3)-iPos(1); iHeight=iPos(4)-iPos(2);
      | iCx=iWidth/2;
      | iCy=iHeight/2;
      | [logoX, logoY] = xlogo(iPos);
      | 
      | 
      | % one time added for param list
      | bo = boolean_output;
      | dblOvrd = dbl_ovrd;
      | precision0 = 1;
      | z0 = [nbits 0 1 1 1];
      | explicitClk = explicit_period;
      | 
      | 
      | % just pass everything to s-function
      | sfcn_mwsv__ = get_param(gcb, 'MaskWSVariables');
      | 
      | nport = get_param(gcbh, 'ports');
      | nin = nport(1);
      | nout = nport(2);
      mask Help: eval('xlWeb(xlhtmldoclink(''Slice''))');
      mask StyleString: popup(Two Bit Locations|Upper Bit Location + Width|Lower Bit Location + Width),edit,edit,popup(LSB of Input|Binary Point of Input|MSB of Input),edit,popup(LSB of Input|Binary Point of Input|MSB of Input),checkbox,checkbox,edit,checkbox
      mask Display:
      | patch([0 iWidth iWidth 0],[0 0 iHeight iHeight] , bg);
      | patch(logoX,logoY , fg);
      | port_label('output',1,'[a:b]');
      | 
      | ;plot([0 0 iWidth iWidth 0], [0 iHeight iHeight 0 0]);
  Sync : S-Function  FunctionName=xldeprecated  Parameters=nin,nout  mask(Xilinx Pipeline Synchronization Block){inputs=2, latency=1, explicit_period=off, period=1, dbl_ovrd=off, show_param=off, xl_area=[0, 0, 0, 0, 0, 0, 0], xl_use_area=off}
      mask prompts: inputs "Number of Channels"; latency "Latency  (minimum per channel)"; explicit_period "Use Explicit Sample Period"; period "Sample Period  (use -1 to inherit first known input period)"; dbl_ovrd "Override with Doubles"; show_param "---------------------- Show Implementation Parameters -----------------------------------------------------------------------------------"; xl_area "FPGA Area [Slices, FFs, BRAMs, LUTs, IOBs, Emb. Mults, TBUFs]"; xl_use_area "Use Area Above For Estimation"
      mask help:
      | BLOCK IS OUT OF DATE.
      |
      | This block is from an outdated copy of the Xilinx Blockset. Please run xlUpdateModel('<model-name>') to update to the latest version.
      mask init:
      | num_inputs = inputs+1;
      | [designRoot, family, part, speed, package, simulinkPeriod, sysclkPeriod, dbl_ovrd, trimVbit] = xlSysgenSettings(gcb,1,1);
      | [bg,fg] = xlcmap_r3('XBlock',dbl_ovrd);
      | iPos = get_param(gcb,'Position');
      | iWidth=iPos(3)-iPos(1); iHeight=iPos(4)-iPos(2);
      | iCx=iWidth/2;
      | iCy=iHeight/2;
      | [logoX, logoY] = xlogo(iPos);
      | zstr='z'; zpstr='-k';
      | if latency > 0
      |   zstr = 'z';
      |   zpstr = sprintf('-k -%d',latency);
      | end
      | zstrx = 0.45*iWidth-3; if (zstrx<3) zstrx=3; end
      | zstry = 0.36*iHeight-7; if (zstry<3) zstry=3; end
      | 
      | % one time added for param list
      | dblOvrd = dbl_ovrd;
      | numInputs = num_inputs;
      | precision0 = 1;
      | precision1 = 1;
      | precision2 = 1;
      | precision3 = 1;
      | explicitClk = explicit_period;
      | 
      | 
      | % just pass everything to s-function
      | sfcn_mwsv__ = get_param(gcb, 'MaskWSVariables');
      | 
      | nport = get_param(gcbh, 'ports');
      | nin = nport(1);
      | nout = nport(2);
      mask Help: eval('xlWeb(xlhtmldoclink(''Sync''))');
      mask StyleString: popup(2|3|4),edit,checkbox,edit,checkbox,checkbox,edit,checkbox
      mask Display:
      | patch([0 iWidth iWidth 0],[0 0 iHeight iHeight] ,bg);
      | patch(logoX,logoY,  fg);
      | text(zstrx,zstry,zstr);
      | text(zstrx+5,zstry+5,zpstr);
      | 
      | ;plot([0 0 iWidth iWidth 0], [0 iHeight iHeight 0 0]);
  Threshold : S-Function  FunctionName=xldeprecated  Parameters=nin,nout  mask(Xilinx Threshold Block){latency=0, explicit_period=off, period=1, en=off, dbl_ovrd=off, show_param=off, xl_area=[0, 0, 0, 0, 0, 0, 0], xl_use_area=off}
      mask prompts: explicit_period "Use Explicit Sample Period"; period "Sample Period  (use -1 to inherit first known input period)"; en "Provide Enable Port"; dbl_ovrd "Override with Doubles"; show_param "---------------------- Show Implementation Parameters -----------------------------------------------------------------------------------"; xl_area "FPGA Area [Slices, FFs, BRAMs, LUTs, IOBs, Emb. Mults, TBUFs]"; xl_use_area "Use Area Above For Estimation"
      mask help:
      | BLOCK IS OUT OF DATE.
      |
      | This block is from an outdated copy of the Xilinx Blockset. Please run xlUpdateModel('<model-name>') to update to the latest version.
      mask init:
      | rst = 0;
      | if(latency > 0)
      |    [enPortNum,enPortStr,rstPortNum,rstPortStr] = xlport_en_rst(en,rst,2);
      | else
      |     [enPortNum,enPortStr,rstPortNum,rstPortStr] = xlport_en_rst(0,0,2);
      | end
      | [designRoot, family, part, speed, package, simulinkPeriod, sysclkPeriod, dbl_ovrd, trimVbit] = xlSysgenSettings(gcb,1,1);
      | zstr='';
      | zpstr='';
      | if latency > 0
      |   zstr = 'z';
      |   zpstr = sprintf('-%d', latency);
      | end
      | [bg,fg] = xlcmap_r3('XBlock',dbl_ovrd);
      | iPos = get_param(gcb,'Position');
      | iWidth=iPos(3)-iPos(1); iHeight=iPos(4)-iPos(2);
      | iCx=iWidth/2;
      | iCy=iHeight/2;
      | [logoX, logoY] = xlogo(iPos);
      | zstrx = 0.45*iWidth-3; if (zstrx<3) zstrx=3; end
      | zstry = 0.36*iHeight-7; if (zstry<3) zstry=3; end
      | 
      | 
      | % one time added for param list
      | dblOvrd = dbl_ovrd;
      | precision0 = 2;
      | z0 = [2  0 2 1 1];
      | explicitClk = explicit_period;
      | hasEN = en;
      | hasRST = rst;
      | 
      | 
      | % just pass everything to s-function
      | sfcn_mwsv__ = get_param(gcb, 'MaskWSVariables');
      | 
      | nport = get_param(gcbh, 'ports');
      | nin = nport(1);
      | nout = nport(2);
      mask Help: eval('xlWeb(xlhtmldoclink(''Threshold''))');
      mask Display:
      | patch([0 iWidth iWidth 0],[0 0 iHeight iHeight] , bg);
      | patch(logoX,logoY , fg);
      | text(zstrx,zstry,zstr);
      | text(zstrx+5,zstry+5,zpstr);
      | port_label('output',1,'sgn');
      | port_label('input',enPortNum,enPortStr);
      | ;plot([0 0 iWidth iWidth 0], [0 iHeight iHeight 0 0]);
  Time Division Demultiplexer : S-Function  FunctionName=xldeprecated  Parameters=nin,nout  mask(Xilinx Time Division Demultiplexer Block){frame_pattern=[1 1 1 1], impl_style=Multiple Channel, explicit_period=off, period=1, vin=off, dbl_ovrd=off, show_param=off, xl_area=[0, 0, 0, 0, 0, 0, 0], xl_use_area=off}
      mask prompts: frame_pattern "Frame Sampling Pattern (example: [1 0 1 0])"; impl_style "Implementation"; explicit_period "Use Explicit Sample Period"; period "Sample Period  (use -1 to inherit first known input period)"; vin "Provide Valid Port"; dbl_ovrd "Override with Doubles"; show_param "---------------------- Show Implementation Parameters -----------------------------------------------------------------------------------"; xl_area "FPGA Area [Slices, FFs, BRAMs, LUTs, IOBs, Emb. Mults, TBUFs]"; xl_use_area "Use Area Above For Estimation"
      mask help:
      | BLOCK IS OUT OF DATE.
      |
      | This block is from an outdated copy of the Xilinx Blockset. Please run xlUpdateModel('<model-name>') to update to the latest version.
      mask init:
      | fp = zeros(1,32);
      | frame_size = max(size(frame_pattern));
      | fp(1:frame_size) = frame_pattern;
      | num_outputs = sum(frame_pattern);
      | if  ( find((frame_pattern~=1) & (frame_pattern~=0)))
      |     frame_pattern = 'error';
      | else
      |  frame_pattern = char( (frame_pattern ~= 0) + 48 );
      | end;
      | 
      | vinPortNum = 1;
      | vinPortStr = '';
      | voutPortNum = 1;
      | voutPortStr = '';
      | 
      | [designRoot, family, part, speed, package, simulinkPeriod, sysclkPeriod, dbl_ovrd, trimVbit] = xlSysgenSettings(gcb,1,1);
      | [bg,fg] = xlcmap_r3('XBlock',dbl_ovrd);
      | iPos = get_param(gcb,'Position');
      | iWidth=iPos(3)-iPos(1); iHeight=iPos(4)-iPos(2);
      | iCx=iWidth/2;
      | iCy=iHeight/2;
      | [logoX, logoY] = xlogo(iPos);
      | 
      | 
      | dprt = ones(1,32);
      | dstr0 = ''; dstr1 = ''; dstr2='';dstr3='';dstr4='';dstr5='';dstr6='';dstr7='';dstr8='';dstr9='';
      | dstr10='';dstr11='';dstr12='';dstr12='';dstr13='';dstr14='';dstr15='';dstr16='';dstr17='';
      | dstr18='';dstr19='';dstr20='';dstr21='';dstr22='';dstr23='';dstr24='';dstr25='';dstr26='';
      | dstr27='';dstr28='';dstr29='';dstr30='';dstr31='';
      | 
      | if (impl_style ==1)
      | 	str = sprintf(' %d',frame_size/num_outputs);
      | 	dstr0 = 'q';
      | 	num_outputs = 1;
      | 	latency =1;
      | else
      | 	str = sprintf(' %d',frame_size);
      | 	latency = 0;
      | 	num_outputs = 0;
      | 	for i =1:frame_size
      |     	if (fp(i) == 1)
      | 			num_outputs = num_outputs + 1;
      | 			dprt(i) = num_outputs;
      |     	end
      |  	end
      | 	if (fp(1)==1) dstr0 ='q0'; end
      | 	if (fp(2)==1) dstr1 ='q1'; end
      | 	if (fp(3)==1) dstr2 ='q2'; end
      | 	if (fp(4)==1) dstr3 ='q3'; end
      | 	if (fp(5)==1) dstr4 ='q4'; end
      | 	if (fp(6)==1) dstr5 ='q5'; end
      | 	if (fp(7)==1) dstr6 ='q6'; end
      | 	if (fp(8)==1) dstr7 ='q7'; end
      | 	if (fp(9)==1) dstr8 ='q8'; end
      | 	if (fp(10)==1) dstr9 ='q9'; end
      | 	if (fp(11)==1) dstr10 ='q10'; end
      | 	if (fp(12)==1) dstr11 ='q11'; end
      | 	if (fp(13)==1) dstr12 ='q12'; end
      | 	if (fp(14)==1) dstr13 ='q13'; end
      | 	if (fp(15)==1) dstr14 ='q14'; end
      | 	if (fp(16)==1) dstr15 ='q15'; end
      | 	if (fp(17)==1) dstr16 ='q16'; end
      | 	if (fp(18)==1) dstr17 ='q17'; end
      | 	if (fp(19)==1) dstr18 ='q18'; end
      | 	if (fp(20)==1) dstr19 ='q19'; end
      | 	if (fp(21)==1) dstr20 ='q20'; end
      | 	if (fp(22)==1) dstr21 ='q21'; end
      | 	if (fp(23)==1) dstr22 ='q22'; end
      | 	if (fp(24)==1) dstr23 ='q23'; end
      | 	if (fp(25)==1) dstr24 ='q24'; end
      | 	if (fp(26)==1) dstr25 ='q25'; end
      | 	if (fp(27)==1) dstr26 ='q26'; end
      | 	if (fp(28)==1) dstr27 ='q27'; end
      | 	if (fp(29)==1) dstr28 ='q28'; end
      | 	if (fp(30)==1) dstr29 ='q29'; end
      | 	if (fp(31)==1) dstr30 ='q30'; end
      | 	if (fp(32)==1) dstr31 ='q31'; end
      | end
      | 
      | if (vin==1)
      | 	num_outputs = num_outputs+1;
      | 	voutPortNum = num_outputs;
      | 	voutPortStr = 'vout';
      | 	vinPortNum = 2;
      | 	vinPortStr = 'vin';
      | end
      | 
      | % one time added for param list
      | precision0 = 1;
      | precision1 = 1;
      | precision2 = 1;
      | precision3 = 1;
      | precision4 = 1;
      | precision5 = 1;
      | precision6 = 1;
      | precision7 = 1;
      | precision8 = 1;
      | precision9 = 1;
      | precision10 = 1;
      | precision11 = 1;
      | precision12 = 1;
      | precision13 = 1;
      | precision14 = 1;
      | precision15 = 1;
      | precision16 = 1;
      | precision17 = 1;
      | precision18 = 1;
      | precision19 = 1;
      | precision20 = 1;
      | precision21 = 1;
      | precision22 = 1;
      | precision23 = 1;
      | precision24 = 1;
      | precision25 = 1;
      | precision26 = 1;
      | precision27 = 1;
      | precision28 = 1;
      | precision29 = 1;
      | precision30 = 1;
      | precision31 = 1;
      | precision32 = 1;
      | 
      | dblOvrd = dbl_ovrd;
      | explicitClk = explicit_period;
      | 
      | clear fp;
      | 
      | aw = 3;
      | ah = 7;
      | arrowX = [0 (-aw) (-aw) 0 0 (1) (1) (aw+1) (aw+1) (1)];
      | arrowY = [(ah-1) (ah-aw-1) (ah-aw) (ah) (-ah) (-ah) (ah) (ah-aw) (ah-aw-1) (ah-1)];
      | arrowX = arrowX + iCx - 2 - 3.5*length(str);
      | arrowY = iCy - arrowY + 2;
      | zstrx = 0.45*iWidth-3; if (zstrx<3) zstrx=3; end
      | zstry = 0.36*iHeight-7; if (zstry<3) zstry=3; end
      | zstr='z';
      | zpstr='';
      | if (impl_style ==1)
      |   zpstr = sprintf('-%d', 2);
      | else
      |   zpstr = sprintf('-%d', 1+vin);	
      | end
      | 
      | % just pass everything to s-function
      | sfcn_mwsv__ = get_param(gcb, 'MaskWSVariables');
      | 
      | nport = get_param(gcbh, 'ports');
      | nin = nport(1);
      | nout = nport(2);
      mask Help: eval('xlWeb(xlhtmldoclink(''Time Division Demultiplexer''))');
      mask StyleString: edit,popup(Single Channel|Multiple Channel),checkbox,edit,checkbox,checkbox,checkbox,edit,checkbox
      mask Display:
      | patch([0 iWidth iWidth 0],[0 0 iHeight iHeight] , bg);
      | patch(logoX,logoY, fg);
      | plot(arrowX,arrowY);
      | disp(str);
      | text(zstrx,zstry,zstr);
      | text(zstrx+5,zstry+5,zpstr);
      | port_label('input',1,'d');
      | port_label('input',vinPortNum,vinPortStr);
      | port_label('output',dprt(2),dstr1);
      | port_label('output',dprt(3),dstr2);
      | port_label('output',dprt(4),dstr3);
      | port_label('output',dprt(5),dstr4);
      | port_label('output',dprt(6),dstr5);
      | port_label('output',dprt(7),dstr6);
      | port_label('output',dprt(8),dstr7);
      | port_label('output',dprt(9),dstr8);
      | port_label('output',dprt(10),dstr9);
      | port_label('output',dprt(11),dstr10);
      | port_label('output',dprt(12),dstr11);
      | port_label('output',dprt(13),dstr12);
      | port_label('output',dprt(14),dstr13);
      | port_label('output',dprt(15),dstr14);
      | port_label('output',dprt(16),dstr15);
      | port_label('output',dprt(17),dstr16);
      | port_label('output',dprt(18),dstr17);
      | port_label('output',dprt(19),dstr18);
      | port_label('output',dprt(20),dstr19);
      | port_label('output',dprt(21),dstr20);
      | port_label('output',dprt(22),dstr21);
      | port_label('output',dprt(23),dstr22);
      | port_label('output',dprt(24),dstr23);
      | port_label('output',dprt(25),dstr24);
      | port_label('output',dprt(26),dstr25);
      | port_label('output',dprt(27),dstr26);
      | port_label('output',dprt(28),dstr27);
      | port_label('output',dprt(29),dstr28);
      | port_label('output',dprt(30),dstr29);
      | port_label('output',dprt(31),dstr30);
      | port_label('output',dprt(32),dstr31);
      | port_label('output',voutPortNum,voutPortStr);
      | port_label('output',dprt(1),dstr0);
      | ;plot([0 0 iWidth iWidth 0], [0 iHeight iHeight 0 0]);
  Time Division Multiplexer : S-Function  FunctionName=xldeprecated  Parameters=nin,nout  mask(Xilinx Time Division Multiplexer Block){inputs=4, explicit_period=off, period=1, vin=off, dbl_ovrd=off, show_param=off, xl_area=[0, 0, 0, 0, 0, 0, 0], xl_use_area=off}
      mask prompts: inputs "Number of Inputs"; explicit_period "Use Explicit Sample Period"; period "Sample Period  (use -1 to inherit first known input period)"; vin "Provide Valid Port"; dbl_ovrd "Override with Doubles"; show_param "---------------------- Show Implementation Parameters -----------------------------------------------------------------------------------"; xl_area "FPGA Area [Slices, FFs, BRAMs, LUTs, IOBs, Emb. Mults, TBUFs]"; xl_use_area "Use Area Above For Estimation"
      mask help:
      | BLOCK IS OUT OF DATE.
      |
      | This block is from an outdated copy of the Xilinx Blockset. Please run xlUpdateModel('<model-name>') to update to the latest version.
      mask init:
      | [designRoot, family, part, speed, package, simulinkPeriod, sysclkPeriod, dbl_ovrd, trimVbit] = xlSysgenSettings(gcb,1,1);
      | [bg,fg] = xlcmap_r3('XBlock',dbl_ovrd);
      | iPos = get_param(gcb,'Position');
      | iWidth=iPos(3)-iPos(1); iHeight=iPos(4)-iPos(2);
      | iCx=iWidth/2;
      | iCy=iHeight/2;
      | [logoX, logoY] = xlogo(iPos);
      | inputs=inputs+1;
      | str = sprintf(' %d',inputs);
      | aw = 3;
      | ah = 7;
      | arrowX = [0 (-aw) (-aw) 0 0 (1) (1) (aw+1) (aw+1) (1)];
      | arrowY = [(ah-1) (ah-aw-1) (ah-aw) (ah) (-ah) (-ah) (ah) (ah-aw) (ah-aw-1) (ah-1)];
      | arrowX = arrowX + iCx - 1 - 3.5*length(str);
      | arrowY = arrowY + iCy + 3;
      | 
      | latency=0;
      | dprt = [1:inputs 1+zeros(1,32-inputs)];
      | dstr0 = 'd0';
      | dstr1 = 'd1';
      | dstr2='';dstr3='';dstr4='';dstr5='';dstr6='';dstr7='';dstr8='';dstr9='';dstr10='';
      | dstr11='';dstr12='';dstr12='';dstr13='';dstr14='';dstr15='';dstr16='';dstr17='';dstr18='';dstr19='';dstr20='';dstr21='';dstr22='';dstr23='';dstr24='';dstr25='';dstr26='';dstr27='';dstr28='';dstr29='';dstr30='';dstr31='';
      | 
      | if (inputs>2) dstr2 = 'd2'; end
      | if (inputs>3) dstr3 = 'd3'; end
      | if (inputs>4) dstr4 = 'd4'; end
      | if (inputs>5) dstr5 = 'd5'; end
      | if (inputs>6) dstr6 = 'd6'; end
      | if (inputs>7) dstr7 = 'd7'; end
      | if (inputs>8) dstr8 = 'd8'; end
      | if (inputs>9) dstr9 = 'd9'; end
      | if (inputs>10) dstr10 = 'd10'; end
      | if (inputs>11) dstr11 = 'd11'; end
      | if (inputs>12) dstr12 = 'd12'; end
      | if (inputs>13) dstr13 = 'd13'; end
      | if (inputs>14) dstr14 = 'd14'; end
      | if (inputs>15) dstr15 = 'd15'; end
      | if (inputs>16) dstr16 = 'd16'; end
      | if (inputs>17) dstr17 = 'd17'; end
      | if (inputs>18) dstr18 = 'd18'; end
      | if (inputs>19) dstr19 = 'd19'; end
      | if (inputs>20) dstr20 = 'd20'; end
      | if (inputs>21) dstr21 = 'd21'; end
      | if (inputs>22) dstr22 = 'd22'; end
      | if (inputs>23) dstr23 = 'd23'; end
      | if (inputs>24) dstr24 = 'd24'; end
      | if (inputs>25) dstr25 = 'd25'; end
      | if (inputs>26) dstr26 = 'd26'; end
      | if (inputs>27) dstr27 = 'd27'; end
      | if (inputs>28) dstr28 = 'd28'; end
      | if (inputs>29) dstr29 = 'd29'; end
      | if (inputs>30) dstr30 = 'd30'; end
      | if (inputs>31) dstr31 = 'd31'; end
      | 
      | vinPortNum = 1;
      | vinPortStr = '';
      | voutPortNum = 1;
      | voutPortStr = '';
      | if (vin==1)
      | 	voutPortNum = 2;
      | 	voutPortStr = 'vout';
      | 	vinPortNum = inputs+1;
      | 	vinPortStr = 'vin';
      | end
      | 
      | % one time added for param list
      | precision0 = 1;
      | precision1 = 1;
      | 
      | dblOvrd = dbl_ovrd;
      | explicitClk = explicit_period;
      | 
      | % just pass everything to s-function
      | sfcn_mwsv__ = get_param(gcb, 'MaskWSVariables');
      | 
      | nport = get_param(gcbh, 'ports');
      | nin = nport(1);
      | nout = nport(2);
      mask Help: eval('xlWeb(xlhtmldoclink(''Time Division Multiplexer''))');
      mask StyleString: popup(2|3|4|5|6|7|8|9|10|11|12|13|14|15|16|17|18|19|20|21|22|23|24|25|26|27|28|29|30|31|32),checkbox,edit,checkbox,checkbox,checkbox,edit,checkbox
      mask Display:
      | patch([0 iWidth iWidth 0],[0 0 iHeight iHeight] , bg);
      | patch(logoX,logoY, fg);
      | plot(arrowX,arrowY);
      | disp(str);
      | port_label('input',vinPortNum,vinPortStr);
      | port_label('input',dprt(2),dstr1);
      | port_label('input',dprt(3),dstr2);
      | port_label('input',dprt(4),dstr3);
      | port_label('input',dprt(5),dstr4);
      | port_label('input',dprt(6),dstr5);
      | port_label('input',dprt(7),dstr6);
      | port_label('input',dprt(8),dstr7);
      | port_label('input',dprt(9),dstr8);
      | port_label('input',dprt(10),dstr9);
      | port_label('input',dprt(11),dstr10);
      | port_label('input',dprt(12),dstr11);
      | port_label('input',dprt(13),dstr12);
      | port_label('input',dprt(14),dstr13);
      | port_label('input',dprt(15),dstr14);
      | port_label('input',dprt(16),dstr15);
      | port_label('input',dprt(17),dstr16);
      | port_label('input',dprt(18),dstr17);
      | port_label('input',dprt(19),dstr18);
      | port_label('input',dprt(20),dstr19);
      | port_label('input',dprt(21),dstr20);
      | port_label('input',dprt(22),dstr21);
      | port_label('input',dprt(23),dstr22);
      | port_label('input',dprt(24),dstr23);
      | port_label('input',dprt(25),dstr24);
      | port_label('input',dprt(26),dstr25);
      | port_label('input',dprt(27),dstr26);
      | port_label('input',dprt(28),dstr27);
      | port_label('input',dprt(29),dstr28);
      | port_label('input',dprt(30),dstr29);
      | port_label('input',dprt(31),dstr30);
      | port_label('input',dprt(32),dstr31);
      | port_label('output',voutPortNum,voutPortStr);
      | port_label('output',1,'q');
      | port_label('input',dprt(1),dstr0);
      | port_label('input',dprt(2),dstr1);
      | ;plot([0 0 iWidth iWidth 0], [0 iHeight iHeight 0 0]);
  To FIFO : S-Function  FunctionName=xldeprecated  Parameters=nin,nout  mask(Xilinx Shared Memory Based To FIFO){shared_memory_name='Bar', depth=16, percent_nbits=1, explicit_period=off, period=1, dbl_ovrd=off, show_param=off, mem_type=Block RAM, xl_area=[0, 0, 0, 0, 0, 0, 0], xl_use_area=off, core_version=1.1}
      mask prompts: shared_memory_name "Shared Memory Name"; percent_nbits "Bits of Precision to Use for "Percent Full" Signal"; explicit_period "Use Explicit Sample Period"; period "Sample Period  (use -1 to inherit first known input period)"; dbl_ovrd "Override with Doubles"; show_param "---------------------- Show Implementation Parameters -----------------------------------------------------------------------------------"; mem_type "Memory Type"; xl_area "FPGA Area [Slices, FFs, BRAMs, LUTs, IOBs, Emb. Mults, TBUFs]"; xl_use_area "Use Area Above For Estimation"; core_version "Core Version"
      mask help:
      | BLOCK IS OUT OF DATE.
      |
      | This block is from an outdated copy of the Xilinx Blockset. Please run xlUpdateModel('<model-name>') to update to the latest version.
      mask init:
      | edepth = 2^(3+depth);
      | 
      | dmem = mem_type - 1;
      | [designRoot, family, part, speed, package, simulinkPeriod, sysclkPeriod, dbl_ovrd, trimVbit] = xlSysgenSettings(gcb,1,1);
      | [bg,fg] = xlcmap_r3('Shmem',dbl_ovrd);
      | iPos = get_param(gcb,'Position');
      | iWidth=iPos(3)-iPos(1); iHeight=iPos(4)-iPos(2);
      | iCx=iWidth/2;
      | iCy=iHeight/2;
      | [logoX, logoY] = xlogo(iPos);
      | % one time added for param list
      | countWidth = sscanf(percent_nbits,'%f');
      | latency = 1;
      | dblOvrd = dbl_ovrd;
      | useCore = 1;
      | precision0 = 1;
      | precision1 = 1;
      | precision2 = 1;
      | precision3 = 1;
      | z1 = [countWidth countWidth 1 1 1];
      | depth = edepth;
      | explicitClk = explicit_period;
      | 
      | % just pass everything to s-function
      | sfcn_mwsv__ = get_param(gcb, 'MaskWSVariables');
      | 
      | nport = get_param(gcbh, 'ports');
      | nin = nport(1);
      | nout = nport(2);
      settings: AttributesFormatString=<< %<shared_memory_name> >>
      mask Help: eval('xlWeb(xlhtmldoclink(''To FIFO''))');
      mask StyleString: edit,popup(16|32|64|128|256|512|1K|2K|4K|8K|16K|32K|64K),popup(1|2|3|4|5|6|7|8|9|10),checkbox,edit,checkbox,checkbox,popup(Block RAM|Distributed RAM|FIFO16),edit,checkbox,edit
      mask Display:
      | patch([0 iWidth iWidth 0],[0 0 iHeight iHeight] , bg);
      | patch(logoX,logoY , fg);
      | 
      | port_label('input',1,'din');
      | port_label('input',2,'we');
      | port_label('output',1,'%full');
      | port_label('output',2,'full');
      | 
      | plot([0 0 iWidth iWidth 0], [0 iHeight iHeight 0 0]);
  To Register : S-Function  FunctionName=xldeprecated  Parameters=nin,nout  mask(Xilinx Shared Memory based To Register){shared_memory_name='Bar', init=0, explicit_period=off, period=1, dbl_ovrd=off, show_param=off, xl_area=[0, 0, 0, 0, 0, 0, 0], xl_use_area=off}
      mask prompts: shared_memory_name "Shared Memory Name"; init "Initial Value"; explicit_period "Use Explicit Sample Period"; period "Sample Period  (use -1 to inherit first known input period)"; dbl_ovrd "Override with Doubles"; show_param "---------------------- Show Implementation Parameters -----------------------------------------------------------------------------------"; xl_area "FPGA Area [Slices, FFs, BRAMs, LUTs, IOBs, Emb. Mults, TBUFs]"; xl_use_area "Use Area Above For Estimation"
      mask help:
      | BLOCK IS OUT OF DATE.
      |
      | This block is from an outdated copy of the Xilinx Blockset. Please run xlUpdateModel('<model-name>') to update to the latest version.
      mask init:
      | [designRoot, family, part, speed, package, simulinkPeriod, sysclkPeriod, dbl_ovrd, trimVbit] = xlSysgenSettings(gcb,1,1);
      | [bg,fg] = xlcmap_r3('Shmem',dbl_ovrd);
      | iPos = get_param(gcb,'Position');
      | iWidth=iPos(3)-iPos(1); iHeight=iPos(4)-iPos(2);
      | iCx=iWidth/2;
      | iCy=iHeight/2;
      | [logoX, logoY] = xlogo(iPos);
      | % one time added for param list
      | latency = 1;
      | dblOvrd = dbl_ovrd;
      | useCore = 1;
      | precision0 = 1;
      | explicitClk = explicit_period;
      | 
      | % just pass everything to s-function
      | sfcn_mwsv__ = get_param(gcb, 'MaskWSVariables');
      | 
      | nport = get_param(gcbh, 'ports');
      | nin = nport(1);
      | nout = nport(2);
      settings: AttributesFormatString=<< %<shared_memory_name> >>
      mask Help: eval('xlWeb(xlhtmldoclink(''To Register''))');
      mask Display:
      | patch([0 iWidth iWidth 0],[0 0 iHeight iHeight] , bg);
      | patch(logoX,logoY , fg);
      | 
      | port_label('input',1,'din');
      | port_label('input',2,'en');
      | port_label('output',1,'dout');
      | 
      | plot([0 0 iWidth iWidth 0], [0 iHeight iHeight 0 0]);
  Toolbar : Subsystem  mask(Xilinx Toolbar){func=xltoolbar}
      mask prompts: func "Launch function"
      mask help: Double click to launch the Xilinx Toolbar.
      mask init:
      | [bg, fg] = xlcmap_r3('XTool');
      | 
      | iPos = get_param(gcb,'Position');
      | iWidth=iPos(3)-iPos(1); iHeight=iPos(4)-iPos(2);
      | iCx=iWidth/2;
      | iCy=iHeight/2;
      | [logoX, logoY] = xlogo(iPos);
      settings: OpenFcn=modelName = get_param(bdroot, 'name');h = errordlg(sprintf(['This block is from an outdated copy of the Xilinx Blockset.\nPlease run xlUpdateModel(''' modelName ''') to update this design.']), 'Update Required');
      mask Help: eval('xlWeb(xlhtmldoclink(''Toolbar''))');
      mask Display:
      | patch([0 iWidth iWidth 0],[0 0 iHeight iHeight] , bg);
      | patch(logoX,logoY , fg);
      | plot([0 0 iWidth iWidth 0], [0 iHeight iHeight 0 0]);
  Up Sample : S-Function  FunctionName=xldeprecated  Parameters=nin,nout  mask(Xilinx Up Sampling Block){sample_ratio=2, copy_samples=off, dbl_ovrd=off, show_param=off, xl_area=[0, 0, 0, 0, 0, 0, 0], xl_use_area=off}
      mask prompts: sample_ratio "Sampling Rate (number of output samples per input sample)"; copy_samples "Copy Samples (otherwise zeros are inserted)"; dbl_ovrd "Override with Doubles"; show_param "---------------------- Show Implementation Parameters -----------------------------------------------------------------------------------"; xl_area "FPGA Area [Slices, FFs, BRAMs, LUTs, IOBs, Emb. Mults, TBUFs]"; xl_use_area "Use Area Above For Estimation"
      mask help:
      | BLOCK IS OUT OF DATE.
      |
      | This block is from an outdated copy of the Xilinx Blockset. Please run xlUpdateModel('<model-name>') to update to the latest version.
      mask init:
      | str = sprintf(' %d',floor(sample_ratio));
      | [designRoot, family, part, speed, package, simulinkPeriod, sysclkPeriod, dbl_ovrd, trimVbit] = xlSysgenSettings(gcb,1,1);
      | [bg,fg] = xlcmap_r3('XBlock',dbl_ovrd);
      | iPos = get_param(gcb,'Position');
      | iWidth=iPos(3)-iPos(1); iHeight=iPos(4)-iPos(2);
      | iCx=iWidth/2;
